simulink model "ACFTsim"  (R2024b)
settings: Solver=ode1  StartTime=0.0  StopTime=inf  FixedStep=0.01  RelTol=1e-3
model workspace (MAT data in the model file):
  op_trim1 = opcond.OperatingReport
  op_trim1.Outputs_(1) = opcond.OutputReport
  op_trim1.Outputs_(1).yspec_ = 0
  op_trim1.Outputs_(1).Block_ = 'ACFT/Mach'
  op_trim1.Outputs_(1).PortWidth_ = 1
  op_trim1.Outputs_(1).PortNumber_ = NaN
  op_trim1.Outputs_(1).y_ = 0.293890617808
  op_trim1.Outputs_(1).Known_ = 0
  op_trim1.Outputs_(1).Min_ = -Inf
  op_trim1.Outputs_(1).Max_ = Inf
  op_trim1.Outputs_(2) = opcond.OutputReport
  op_trim1.Outputs_(2).yspec_ = 0
  op_trim1.Outputs_(2).Block_ = 'ACFT/Beta_deg'
  op_trim1.Outputs_(2).PortWidth_ = 1
  op_trim1.Outputs_(2).PortNumber_ = NaN
  op_trim1.Outputs_(2).Known_ = 1
  op_trim1.Outputs_(2).Min_ = -Inf
  op_trim1.Outputs_(2).Max_ = Inf
  op_trim1.Outputs_(3) = opcond.OutputReport
  op_trim1.Outputs_(3).yspec_ = 0
  op_trim1.Outputs_(3).Block_ = 'ACFT/Alpha_deg'
  op_trim1.Outputs_(3).PortWidth_ = 1
  op_trim1.Outputs_(3).PortNumber_ = NaN
  op_trim1.Outputs_(3).Known_ = 0
  op_trim1.Outputs_(3).Min_ = -Inf
  op_trim1.Outputs_(3).Max_ = Inf
  op_trim1.Outputs_(4) = opcond.OutputReport
  op_trim1.Outputs_(4).yspec_ = 200
  op_trim1.Outputs_(4).Block_ = 'ACFT/Cas_kt'
  op_trim1.Outputs_(4).PortWidth_ = 1
  op_trim1.Outputs_(4).PortNumber_ = NaN
  op_trim1.Outputs_(4).y_ = 194.38408042
  op_trim1.Outputs_(4).Known_ = 1
  op_trim1.Outputs_(4).Min_ = -Inf
  op_trim1.Outputs_(4).Max_ = Inf
  op_trim1.Outputs_(5) = opcond.OutputReport
  op_trim1.Outputs_(5).yspec_ = 0
  op_trim1.Outputs_(5).Block_ = 'ACFT/u_mps'
  op_trim1.Outputs_(5).PortWidth_ = 1
  op_trim1.Outputs_(5).PortNumber_ = NaN
  op_trim1.Outputs_(5).y_ = 100
  op_trim1.Outputs_(5).Known_ = 0
  op_trim1.Outputs_(5).Min_ = -Inf
  op_trim1.Outputs_(5).Max_ = Inf
  op_trim1.Outputs_(6) = opcond.OutputReport
  op_trim1.Outputs_(6).yspec_ = 0
  op_trim1.Outputs_(6).Block_ = 'ACFT/v_mps'
  op_trim1.Outputs_(6).PortWidth_ = 1
  op_trim1.Outputs_(6).PortNumber_ = NaN
  op_trim1.Outputs_(6).Known_ = 0
  op_trim1.Outputs_(6).Min_ = -Inf
  op_trim1.Outputs_(6).Max_ = Inf
  op_trim1.Outputs_(7) = opcond.OutputReport
  op_trim1.Outputs_(7).yspec_ = 0
  op_trim1.Outputs_(7).Block_ = 'ACFT/w_mps'
  op_trim1.Outputs_(7).PortWidth_ = 1
  op_trim1.Outputs_(7).PortNumber_ = NaN
  op_trim1.Outputs_(7).Known_ = 0
  op_trim1.Outputs_(7).Min_ = -Inf
  op_trim1.Outputs_(7).Max_ = Inf
  op_trim1.Outputs_(8) = opcond.OutputReport
  op_trim1.Outputs_(8).yspec_ = 0
  op_trim1.Outputs_(8).Block_ = 'ACFT/phi_deg'
  op_trim1.Outputs_(8).PortWidth_ = 1
  op_trim1.Outputs_(8).PortNumber_ = NaN
  op_trim1.Outputs_(8).Known_ = 0
  op_trim1.Outputs_(8).Min_ = -Inf
  op_trim1.Outputs_(8).Max_ = Inf
  op_trim1.Outputs_(9) = opcond.OutputReport
  op_trim1.Outputs_(9).yspec_ = 0
  op_trim1.Outputs_(9).Block_ = 'ACFT/theta_deg'
  op_trim1.Outputs_(9).PortWidth_ = 1
  op_trim1.Outputs_(9).PortNumber_ = NaN
  op_trim1.Outputs_(9).Known_ = 0
  op_trim1.Outputs_(9).Min_ = -Inf
  op_trim1.Outputs_(9).Max_ = Inf
  op_trim1.Outputs_(10) = opcond.OutputReport
  op_trim1.Outputs_(10).yspec_ = 0
  op_trim1.Outputs_(10).Block_ = 'ACFT/psi_deg'
  op_trim1.Outputs_(10).PortWidth_ = 1
  op_trim1.Outputs_(10).PortNumber_ = NaN
  op_trim1.Outputs_(10).Known_ = 0
  op_trim1.Outputs_(10).Min_ = -Inf
  op_trim1.Outputs_(10).Max_ = Inf
  op_trim1.Outputs_(11) = opcond.OutputReport
  op_trim1.Outputs_(11).yspec_ = 0
  op_trim1.Outputs_(11).Block_ = 'ACFT/p_radps'
  op_trim1.Outputs_(11).PortWidth_ = 1
  op_trim1.Outputs_(11).PortNumber_ = NaN
  op_trim1.Outputs_(11).Known_ = 0
  op_trim1.Outputs_(11).Min_ = -Inf
  op_trim1.Outputs_(11).Max_ = Inf
  op_trim1.Outputs_(12) = opcond.OutputReport
  op_trim1.Outputs_(12).yspec_ = 0
  op_trim1.Outputs_(12).Block_ = 'ACFT/q_radps'
  op_trim1.Outputs_(12).PortWidth_ = 1
  op_trim1.Outputs_(12).PortNumber_ = NaN
  op_trim1.Outputs_(12).Known_ = 0
  op_trim1.Outputs_(12).Min_ = -Inf
  op_trim1.Outputs_(12).Max_ = Inf
  op_trim1.Outputs_(13) = opcond.OutputReport
  op_trim1.Outputs_(13).yspec_ = 0
  op_trim1.Outputs_(13).Block_ = 'ACFT/r_radps'
  op_trim1.Outputs_(13).PortWidth_ = 1
  op_trim1.Outputs_(13).PortNumber_ = NaN
  op_trim1.Outputs_(13).Known_ = 0
  op_trim1.Outputs_(13).Min_ = -Inf
  op_trim1.Outputs_(13).Max_ = Inf
  op_trim1.Outputs_(14) = opcond.OutputReport
  op_trim1.Outputs_(14).yspec_ = 0
  op_trim1.Outputs_(14).Block_ = 'ACFT/x_m'
  op_trim1.Outputs_(14).PortWidth_ = 1
  op_trim1.Outputs_(14).PortNumber_ = NaN
  op_trim1.Outputs_(14).Known_ = 0
  op_trim1.Outputs_(14).Min_ = -Inf
  op_trim1.Outputs_(14).Max_ = Inf
  op_trim1.Outputs_(15) = opcond.OutputReport
  op_trim1.Outputs_(15).yspec_ = 0
  op_trim1.Outputs_(15).Block_ = 'ACFT/y_m'
  op_trim1.Outputs_(15).PortWidth_ = 1
  op_trim1.Outputs_(15).PortNumber_ = NaN
  op_trim1.Outputs_(15).Known_ = 0
  op_trim1.Outputs_(15).Min_ = -Inf
  op_trim1.Outputs_(15).Max_ = Inf
  op_trim1.Outputs_(16) = opcond.OutputReport
  op_trim1.Outputs_(16).yspec_ = 25000
  op_trim1.Outputs_(16).Block_ = 'ACFT/PressAlt_ft'
  op_trim1.Outputs_(16).PortWidth_ = 1
  op_trim1.Outputs_(16).PortNumber_ = NaN
  op_trim1.Outputs_(16).y_ = 0
  op_trim1.Outputs_(16).Known_ = 1
  op_trim1.Outputs_(16).Min_ = -Inf
  op_trim1.Outputs_(16).Max_ = Inf
  op_trim1.Outputs_(17) = opcond.OutputReport
  op_trim1.Outputs_(17).yspec_ = 0
  op_trim1.Outputs_(17).Block_ = 'ACFT/Gspeed_kt'
  op_trim1.Outputs_(17).PortWidth_ = 1
  op_trim1.Outputs_(17).PortNumber_ = NaN
  op_trim1.Outputs_(17).y_ = 194.384450923
  op_trim1.Outputs_(17).Known_ = 0
  op_trim1.Outputs_(17).Min_ = -Inf
  op_trim1.Outputs_(17).Max_ = Inf
  op_trim1.Outputs_(18) = opcond.OutputReport
  op_trim1.Outputs_(18).yspec_ = 0
  op_trim1.Outputs_(18).Block_ = 'ACFT/Track_deg'
  op_trim1.Outputs_(18).PortWidth_ = 1
  op_trim1.Outputs_(18).PortNumber_ = NaN
  op_trim1.Outputs_(18).Known_ = 0
  op_trim1.Outputs_(18).Min_ = -Inf
  op_trim1.Outputs_(18).Max_ = Inf
  op_trim1.Outputs_(19) = opcond.OutputReport
  op_trim1.Outputs_(19).yspec_ = 0
  op_trim1.Outputs_(19).Block_ = 'ACFT/Gamma_deg'
  op_trim1.Outputs_(19).PortWidth_ = 1
  op_trim1.Outputs_(19).PortNumber_ = NaN
  op_trim1.Outputs_(19).y_ = 0
  op_trim1.Outputs_(19).Known_ = 1
  op_trim1.Outputs_(19).Min_ = -Inf
  op_trim1.Outputs_(19).Max_ = Inf
  op_trim1.Outputs_(20) = opcond.OutputReport
  op_trim1.Outputs_(20).yspec_ = 0
  op_trim1.Outputs_(20).Block_ = 'ACFT/nx'
  op_trim1.Outputs_(20).PortWidth_ = 1
  op_trim1.Outputs_(20).PortNumber_ = NaN
  op_trim1.Outputs_(20).y_ = -0.0431036960178
  op_trim1.Outputs_(20).Known_ = 0
  op_trim1.Outputs_(20).Min_ = -Inf
  op_trim1.Outputs_(20).Max_ = Inf
  op_trim1.Outputs_(21) = opcond.OutputReport
  op_trim1.Outputs_(21).yspec_ = 0
  op_trim1.Outputs_(21).Block_ = 'ACFT/ny'
  op_trim1.Outputs_(21).PortWidth_ = 1
  op_trim1.Outputs_(21).PortNumber_ = NaN
  op_trim1.Outputs_(21).Known_ = 0
  op_trim1.Outputs_(21).Min_ = -Inf
  op_trim1.Outputs_(21).Max_ = Inf
  op_trim1.Outputs_(22) = opcond.OutputReport
  op_trim1.Outputs_(22).yspec_ = 0
  op_trim1.Outputs_(22).Block_ = 'ACFT/nz'
  op_trim1.Outputs_(22).PortWidth_ = 1
  op_trim1.Outputs_(22).PortNumber_ = NaN
  op_trim1.Outputs_(22).y_ = 0.0431036960178
  op_trim1.Outputs_(22).Known_ = 0
  op_trim1.Outputs_(22).Min_ = -Inf
  op_trim1.Outputs_(22).Max_ = Inf
  op_trim1.Outputs_(23) = opcond.OutputReport
  op_trim1.Outputs_(23).yspec_ = 0
  op_trim1.Outputs_(23).Block_ = 'ACFT/Thrust_N'
  op_trim1.Outputs_(23).PortWidth_ = 1
  op_trim1.Outputs_(23).PortNumber_ = NaN
  op_trim1.Outputs_(23).Known_ = 0
  op_trim1.Outputs_(23).Min_ = -Inf
  op_trim1.Outputs_(23).Max_ = Inf
  op_trim1.Outputs_(24) = opcond.OutputReport
  op_trim1.Outputs_(24).yspec_ = 0
  op_trim1.Outputs_(24).Block_ = 'ACFT/Alpha_radps'
  op_trim1.Outputs_(24).PortWidth_ = 1
  op_trim1.Outputs_(24).PortNumber_ = NaN
  op_trim1.Outputs_(24).Known_ = 0
  op_trim1.Outputs_(24).Min_ = -Inf
  op_trim1.Outputs_(24).Max_ = Inf
  op_trim1.Outputs_(25) = opcond.OutputReport
  op_trim1.Outputs_(25).yspec_ = 0
  op_trim1.Outputs_(25).Block_ = 'ACFT/Tas_kt'
  op_trim1.Outputs_(25).PortWidth_ = 1
  op_trim1.Outputs_(25).PortNumber_ = NaN
  op_trim1.Outputs_(25).y_ = 194.384450923
  op_trim1.Outputs_(25).Known_ = 0
  op_trim1.Outputs_(25).Min_ = -Inf
  op_trim1.Outputs_(25).Max_ = Inf
  op_trim1.TerminationString_ = 'Could not find a solution that satisfies all constraints.  Relax the constraints to find a feasible solution.'
  op_trim1.OptimizationOutput_.iterations = 1
  op_trim1.OptimizationOutput_.funcCount = 16
  op_trim1.OptimizationOutput_.lssteplength = 1
  op_trim1.OptimizationOutput_.stepsize = 0
  op_trim1.OptimizationOutput_.algorithm = 'active-set'
  op_trim1.OptimizationOutput_.firstorderopt = []
  op_trim1.OptimizationOutput_.constrviolation = 25000
  op_trim1.OptimizationOutput_.message = 'Converged to an infeasible point.
    | 
    | fmincon stopped because the size of the current search direction is less than
    | twice the value of the step size tolerance but constraints are not 
    | satisfied to within the value of the constraint tolerance.
    | 
    | <stopping criteria details>
    | 
    | Optimization stopped because the norm of the current search direction , 0.000000e+00,
    | is less than 2*options.StepTolerance = 1.000000e-06, but the maximum constraint
    | violation, 2.500000e+04, exceeds options.ConstraintTolerance = 1.000000e-06.'
  op_trim1.OptimizationOutput_.bestfeasible = []
  op_trim1.OptimizationOutput_.progress = {'<font face="monospaced"; size=3><BR>', 'Optimizing to solve for all desired dx/dt=0, x(k+1)-x(k)=0, and y=ydes.<BR>', ' <BR>', '(Maximum Error)  Block<BR>', ' ---------------------------------------------------------<BR>', '(2.50000e+04) ACFT/PressAlt_ft<BR>', '(2.50000e+04) ACFT/PressAlt_ft<BR>', ' <BR>', 'Could not find a solution that satisfies all constraints.  Relax the constraints to find a feasible solution.<BR>'}
  op_trim1.Model_ = 'ACFT'
  op_trim1.States_(1) = opcond.StateReport
  op_trim1.States_(1).Nx_ = 1
  op_trim1.States_(1).Block_ = 'ACFT/EquationsMotions/BodyRates/p_radps'
  op_trim1.States_(1).SteadyState_ = 1
  op_trim1.States_(1).dxMin_ = -Inf
  op_trim1.States_(1).dxMax_ = Inf
  op_trim1.States_(1).Known_ = 0
  op_trim1.States_(1).Min_ = -Inf
  op_trim1.States_(1).Max_ = Inf
  op_trim1.States_(2) = opcond.StateReport
  op_trim1.States_(2).dx_ = 0.0213648728432
  op_trim1.States_(2).Nx_ = 1
  op_trim1.States_(2).Block_ = 'ACFT/EquationsMotions/BodyRates/q_radps'
  op_trim1.States_(2).SteadyState_ = 1
  op_trim1.States_(2).dxMin_ = -Inf
  op_trim1.States_(2).dxMax_ = Inf
  op_trim1.States_(2).Known_ = 0
  op_trim1.States_(2).Min_ = -Inf
  op_trim1.States_(2).Max_ = Inf
  op_trim1.States_(3) = opcond.StateReport
  op_trim1.States_(3).Nx_ = 1
  op_trim1.States_(3).Block_ = 'ACFT/EquationsMotions/BodyRates/r_radps'
  op_trim1.States_(3).SteadyState_ = 1
  op_trim1.States_(3).dxMin_ = -Inf
  op_trim1.States_(3).dxMax_ = Inf
  op_trim1.States_(3).Known_ = 0
  op_trim1.States_(3).Min_ = -Inf
  op_trim1.States_(3).Max_ = Inf
  op_trim1.States_(4) = opcond.StateReport
  op_trim1.States_(4).dx_ = -0.422702860553
  op_trim1.States_(4).Nx_ = 1
  op_trim1.States_(4).Block_ = 'ACFT/EquationsMotions/BodyVelocities/u_mps'
  op_trim1.States_(4).x_ = 100
  op_trim1.States_(4).SteadyState_ = 1
  op_trim1.States_(4).dxMin_ = -Inf
  op_trim1.States_(4).dxMax_ = Inf
  op_trim1.States_(4).Known_ = 1
  op_trim1.States_(4).Min_ = -Inf
  op_trim1.States_(4).Max_ = Inf
  op_trim1.States_(5) = opcond.StateReport
  op_trim1.States_(5).Nx_ = 1
  op_trim1.States_(5).Block_ = 'ACFT/EquationsMotions/BodyVelocities/v_mps'
  op_trim1.States_(5).SteadyState_ = 1
  op_trim1.States_(5).dxMin_ = -Inf
  op_trim1.States_(5).dxMax_ = Inf
  op_trim1.States_(5).Known_ = 0
  op_trim1.States_(5).Min_ = -Inf
  op_trim1.States_(5).Max_ = Inf
  op_trim1.States_(6) = opcond.StateReport
  op_trim1.States_(6).dx_ = 9.38394713945
  op_trim1.States_(6).Nx_ = 1
  op_trim1.States_(6).Block_ = 'ACFT/EquationsMotions/BodyVelocities/w_mps'
  op_trim1.States_(6).SteadyState_ = 1
  op_trim1.States_(6).dxMin_ = -Inf
  op_trim1.States_(6).dxMax_ = Inf
  op_trim1.States_(6).Known_ = 0
  op_trim1.States_(6).Min_ = -Inf
  op_trim1.States_(6).Max_ = Inf
  op_trim1.States_(7) = opcond.StateReport
  op_trim1.States_(7).dx_ = 100
  op_trim1.States_(7).Nx_ = 1
  op_trim1.States_(7).Block_ = 'ACFT/EquationsMotions/InertialData/XI_m'
  op_trim1.States_(7).SteadyState_ = 0
  op_trim1.States_(7).dxMin_ = -Inf
  op_trim1.States_(7).dxMax_ = Inf
  op_trim1.States_(7).Known_ = 0
  op_trim1.States_(7).Min_ = -Inf
  op_trim1.States_(7).Max_ = Inf
  op_trim1.States_(8) = opcond.StateReport
  op_trim1.States_(8).Nx_ = 1
  op_trim1.States_(8).Block_ = 'ACFT/EquationsMotions/InertialData/YI_m'
  op_trim1.States_(8).SteadyState_ = 0
  op_trim1.States_(8).dxMin_ = -Inf
  op_trim1.States_(8).dxMax_ = Inf
  op_trim1.States_(8).Known_ = 0
  op_trim1.States_(8).Min_ = -Inf
  op_trim1.States_(8).Max_ = Inf
  op_trim1.States_(9) = opcond.StateReport
  op_trim1.States_(9).Nx_ = 1
  op_trim1.States_(9).Block_ = 'ACFT/EquationsMotions/InertialData/ZI_m'
  op_trim1.States_(9).SteadyState_ = 0
  op_trim1.States_(9).dxMin_ = -Inf
  op_trim1.States_(9).dxMax_ = Inf
  op_trim1.States_(9).Known_ = 0
  op_trim1.States_(9).Min_ = -Inf
  op_trim1.States_(9).Max_ = Inf
  op_trim1.States_(10) = opcond.StateReport
  op_trim1.States_(10).Nx_ = 1
  op_trim1.States_(10).Block_ = 'ACFT/EquationsMotions/LBE_EulerAngles_rad/PHI_rad'
  op_trim1.States_(10).SteadyState_ = 1
  op_trim1.States_(10).dxMin_ = -Inf
  op_trim1.States_(10).dxMax_ = Inf
  op_trim1.States_(10).Known_ = 0
  op_trim1.States_(10).Min_ = -Inf
  op_trim1.States_(10).Max_ = Inf
  op_trim1.States_(11) = opcond.StateReport
  op_trim1.States_(11).Nx_ = 1
  op_trim1.States_(11).Block_ = 'ACFT/EquationsMotions/LBE_EulerAngles_rad/PSI_rad'
  op_trim1.States_(11).SteadyState_ = 1
  op_trim1.States_(11).dxMin_ = -Inf
  op_trim1.States_(11).dxMax_ = Inf
  op_trim1.States_(11).Known_ = 0
  op_trim1.States_(11).Min_ = -Inf
  op_trim1.States_(11).Max_ = Inf
  op_trim1.States_(12) = opcond.StateReport
  op_trim1.States_(12).Nx_ = 1
  op_trim1.States_(12).Block_ = 'ACFT/EquationsMotions/LBE_EulerAngles_rad/THETA_rad'
  op_trim1.States_(12).SteadyState_ = 1
  op_trim1.States_(12).dxMin_ = -Inf
  op_trim1.States_(12).dxMax_ = Inf
  op_trim1.States_(12).Known_ = 0
  op_trim1.States_(12).Min_ = -Inf
  op_trim1.States_(12).Max_ = Inf
  op_trim1.Inputs_(1) = opcond.InputReport
  op_trim1.Inputs_(1).Block_ = 'ACFT/Mass_kg'
  op_trim1.Inputs_(1).PortWidth_ = 1
  op_trim1.Inputs_(1).PortDimensions_ = [1 1]
  op_trim1.Inputs_(1).u_ = 15000
  op_trim1.Inputs_(1).Known_ = 1
  op_trim1.Inputs_(1).Min_ = -Inf
  op_trim1.Inputs_(1).Max_ = Inf
  op_trim1.Inputs_(2) = opcond.InputReport
  op_trim1.Inputs_(2).Block_ = 'ACFT/Elevator_deg'
  op_trim1.Inputs_(2).PortWidth_ = 1
  op_trim1.Inputs_(2).PortDimensions_ = [1 1]
  op_trim1.Inputs_(2).Known_ = 0
  op_trim1.Inputs_(2).Min_ = -30
  op_trim1.Inputs_(2).Max_ = 30
  op_trim1.Inputs_(3) = opcond.InputReport
  op_trim1.Inputs_(3).Block_ = 'ACFT/CG_mac'
  op_trim1.Inputs_(3).PortWidth_ = 1
  op_trim1.Inputs_(3).PortDimensions_ = [1 1]
  op_trim1.Inputs_(3).u_ = 0.4
  op_trim1.Inputs_(3).Known_ = 1
  op_trim1.Inputs_(3).Min_ = -Inf
  op_trim1.Inputs_(3).Max_ = Inf
  op_trim1.Inputs_(4) = opcond.InputReport
  op_trim1.Inputs_(4).Block_ = 'ACFT/Throttle_deg'
  op_trim1.Inputs_(4).PortWidth_ = 1
  op_trim1.Inputs_(4).PortDimensions_ = [1 1]
  op_trim1.Inputs_(4).Known_ = 0
  op_trim1.Inputs_(4).Min_ = 0
  op_trim1.Inputs_(4).Max_ = 1
  op_trim1.Inputs_(5) = opcond.InputReport
  op_trim1.Inputs_(5).Block_ = 'ACFT/Rudder_deg'
  op_trim1.Inputs_(5).PortWidth_ = 1
  op_trim1.Inputs_(5).PortDimensions_ = [1 1]
  op_trim1.Inputs_(5).Known_ = 0
  op_trim1.Inputs_(5).Min_ = -30
  op_trim1.Inputs_(5).Max_ = 30
  op_trim1.Inputs_(6) = opcond.InputReport
  op_trim1.Inputs_(6).Block_ = 'ACFT/Wind_x'
  op_trim1.Inputs_(6).PortWidth_ = 1
  op_trim1.Inputs_(6).PortDimensions_ = [1 1]
  op_trim1.Inputs_(6).Known_ = 1
  op_trim1.Inputs_(6).Min_ = -Inf
  op_trim1.Inputs_(6).Max_ = Inf
  op_trim1.Inputs_(7) = opcond.InputReport
  op_trim1.Inputs_(7).Block_ = 'ACFT/Wind_z'
  op_trim1.Inputs_(7).PortWidth_ = 1
  op_trim1.Inputs_(7).PortDimensions_ = [1 1]
  op_trim1.Inputs_(7).Known_ = 1
  op_trim1.Inputs_(7).Min_ = -Inf
  op_trim1.Inputs_(7).Max_ = Inf
  op_trim1.Inputs_(8) = opcond.InputReport
  op_trim1.Inputs_(8).Block_ = 'ACFT/Wind_y'
  op_trim1.Inputs_(8).PortWidth_ = 1
  op_trim1.Inputs_(8).PortDimensions_ = [1 1]
  op_trim1.Inputs_(8).Known_ = 1
  op_trim1.Inputs_(8).Min_ = -Inf
  op_trim1.Inputs_(8).Max_ = Inf
  op_trim1.Inputs_(9) = opcond.InputReport
  op_trim1.Inputs_(9).Block_ = 'ACFT/Aileron_deg'
  op_trim1.Inputs_(9).PortWidth_ = 1
  op_trim1.Inputs_(9).PortDimensions_ = [1 1]
  op_trim1.Inputs_(9).Known_ = 0
  op_trim1.Inputs_(9).Min_ = -40
  op_trim1.Inputs_(9).Max_ = 40
  op_trim4 : opcond.OperatingReport (value not decoded)
  u_mps = 0
values from neighbouring files (symbols this model uses):
  alfa_deg = -1.8    [initACFT_high.m]    (also in init_Cessna.m = 1)
  b = params.b    [Aerodynamics_Coefficient.m]    (also in AeroforcesandMoments.m; ConversionStab2Aero.m = dynP_Pa*CnB; initACFT_high.m = 21; initACFT_low.m = 21)
  c = params.c    [Aerodynamics_Coefficient.m]    (also in AeroforcesandMoments.m; ConversionStab2Aero.m = dynP_Pa*CmB; initACFT_high.m = 2.5; initACFT_low.m = 2.5)
  CD0 = params.CD0    [Aerodynamics_Coefficient.m]    (also in initACFT_high.m = 0.0281; initACFT_low.m = 0.023; init_Cessna.m = 0.027)
  CD_alpha = params.CD_alpha    [Aerodynamics_Coefficient.m]    (also in initACFT_high.m = 0.5157; initACFT_low.m = 0.1318; init_Cessna.m = 0.26)
  CD_elev = params.CD_elev    [Aerodynamics_Coefficient.m]    (also in initACFT_high.m = 0.0178; initACFT_low.m = 0.0178; init_Cessna.m = 0)
  CL0 = params.CL0    [Aerodynamics_Coefficient.m]    (also in initACFT_high.m = 0.209; initACFT_low.m = 0.19; init_Cessna.m = 0.307)
  Cl_ail = -0.0453    [initACFT_high.m]    (also in initACFT_low.m = -0.0516; init_Cessna.m = -0.229)
  CL_alpha = params.CL_alpha    [Aerodynamics_Coefficient.m]    (also in initACFT_high.m = 8.7491; initACFT_low.m = 6.1879; init_Cessna.m = 4.41)
  CL_AlphaDot = params.CL_AlphaDot    [Aerodynamics_Coefficient.m]    (also in initACFT_high.m = 1.27; initACFT_low.m = 1.93; init_Cessna.m = 0)
  Cl_beta = -0.1352    [initACFT_high.m]    (also in initACFT_low.m; init_Cessna.m = -0.0923)
  CL_elev = params.CL_elev    [Aerodynamics_Coefficient.m]    (also in initACFT_high.m = 0.538; initACFT_low.m = 0.4727; init_Cessna.m = 0.43)
  Cl_p = -0.45    [initACFT_high.m]    (also in initACFT_low.m; init_Cessna.m = -0.484)
  CL_q = params.CL_q    [Aerodynamics_Coefficient.m]    (also in initACFT_high.m = 4.14; initACFT_low.m = 4.66; init_Cessna.m = 3.9)
  Cl_r = 0.100    (= 0.1)    [initACFT_high.m]    (also in initACFT_low.m; init_Cessna.m = 0.0798)
  Cl_rud = 0.0333    [initACFT_high.m]    (also in initACFT_low.m = 0.0289; init_Cessna.m = 0.0147)
  Cm0 = params.Cm0    [Aerodynamics_Coefficient.m]    (also in initACFT_high.m = 0; initACFT_low.m = 0.0133; init_Cessna.m = 0.04)
  Cm_alpha = params.Cm_alpha    [Aerodynamics_Coefficient.m]    (also in initACFT_high.m = -2.4351; initACFT_low.m = -2.0168; init_Cessna.m = -0.613)
  Cm_AlphaDot = params.Cm_AlphaDot    [Aerodynamics_Coefficient.m]    (also in initACFT_high.m = -4.53; initACFT_low.m = -6.76; init_Cessna.m = -7.27)
  Cm_elev = params.Cm_elev    [Aerodynamics_Coefficient.m]    (also in initACFT_high.m = -1.9079; initACFT_low.m = -1.6788; init_Cessna.m = -1.122)
  Cm_q = params.Cm_q    [Aerodynamics_Coefficient.m]    (also in initACFT_high.m = -37.6; initACFT_low.m = -36.3; init_Cessna.m = -12.4)
  Cn_ail = -8.5944e-04    (= -0.00085944)    [initACFT_high.m]    (also in initACFT_low.m = -0.00063025; init_Cessna.m = -0.0216)
  Cn_beta = 0.1478    [initACFT_high.m]    (also in initACFT_low.m = 0.1209; init_Cessna.m = 0.0587)
  Cn_p = -0.114    [initACFT_high.m]    (also in initACFT_low.m; init_Cessna.m = -0.0278)
  Cn_r = -0.15    [initACFT_high.m]    (also in initACFT_low.m = -0.3; init_Cessna.m = -0.0937)
  Cn_rud = -0.1100    (= -0.11)    [initACFT_high.m]    (also in initACFT_low.m = -0.102; init_Cessna.m = -0.0645)
  CY_ail = 0    [initACFT_high.m]    (also in initACFT_low.m; init_Cessna.m)
  CY_beta = params.CY_beta    [Aerodynamics_Coefficient.m]    (also in initACFT_high.m = -1.2777; initACFT_low.m = -1.1803; init_Cessna.m = -0.404)
  CY_p = params.CY_p    [Aerodynamics_Coefficient.m]    (also in initACFT_high.m = 0.3; initACFT_low.m = 0.3; init_Cessna.m = -0.075)
  CY_r = params.CY_r    [Aerodynamics_Coefficient.m]    (also in initACFT_high.m = 0.91; initACFT_low.m = 0.91; init_Cessna.m = 0.214)
  CY_rud = params.CY_rud    [Aerodynamics_Coefficient.m]    (also in initACFT_high.m = 0.4343; initACFT_low.m = 0.4016; init_Cessna.m = 0.187)
  g = params.g_mps    [IsaAtmo.m]    (also in extForces.AndMoments.m = params.g; initACFT_high.m = 9.80665; init_Cessna.m = 9.80665)
  Inertia = [Ixx 0 -Ixz; 0 Iyy 0; -Ixz 0 Izz]    [initACFT_high.m]    (also in initACFT_low.m; init_Cessna.m)
  nrho = 0.75    [initACFT_high.m]    (also in initACFT_low.m; init_Cessna.m)
  nv = params.nv    [Propulsion.m]    (also in initACFT_high.m = 0; initACFT_low.m = 0; init_Cessna.m = -1)
  rho_reference_kgpm3 = 1.225    [initACFT_high.m]    (also in init_Cessna.m)
  S = 45    [initACFT_high.m]    (also in initACFT_low.m; init_Cessna.m = 16.2)
  Tmax = params.Tmax    [Propulsion.m]    (also in initACFT_high.m = 68000; initACFT_low.m = 68000; init_Cessna.m = 2070)
  Trimming = 0    [Sim_trim_input.m]    (also in init_Cessna.m)
  V_reference_mps = params.V    [Propulsion.m]    (also in initACFT_high.m = 200; init_Cessna.m = 51.4)
  xf_m = params.xf_m    [Propulsion.m]    (also in initACFT_high.m = -3.8; initACFT_low.m = -3.8; init_Cessna.m = 1)
  y_cg = 0    [initACFT_high.m]    (also in initACFT_low.m; init_Cessna.m)
  z_cg = -0.4    [initACFT_high.m]    (also in initACFT_low.m; init_Cessna.m = 0.2)
  zf_m = params.zf_m    [Propulsion.m]    (also in initACFT_high.m = -0.6; initACFT_low.m = -0.6; init_Cessna.m = 0)
undefined symbols (not defined in the file or in its folder): Earth, Receive, Send, WGS84
libraries: aerolibfltsims x2, vrlib x1, aerolibtransform2 x1
settings Model: PacingRate=0.110000  LastModifiedBy=jogos
settings DataIOCC: ExternalInput=getinputstruct(op_trim4)  InitialState=getstatestruct(op_trim4)

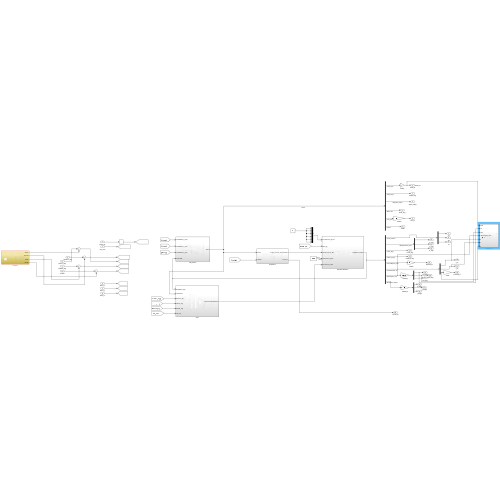
[thumbnail: Simulink's stored preview of the top-level diagram]
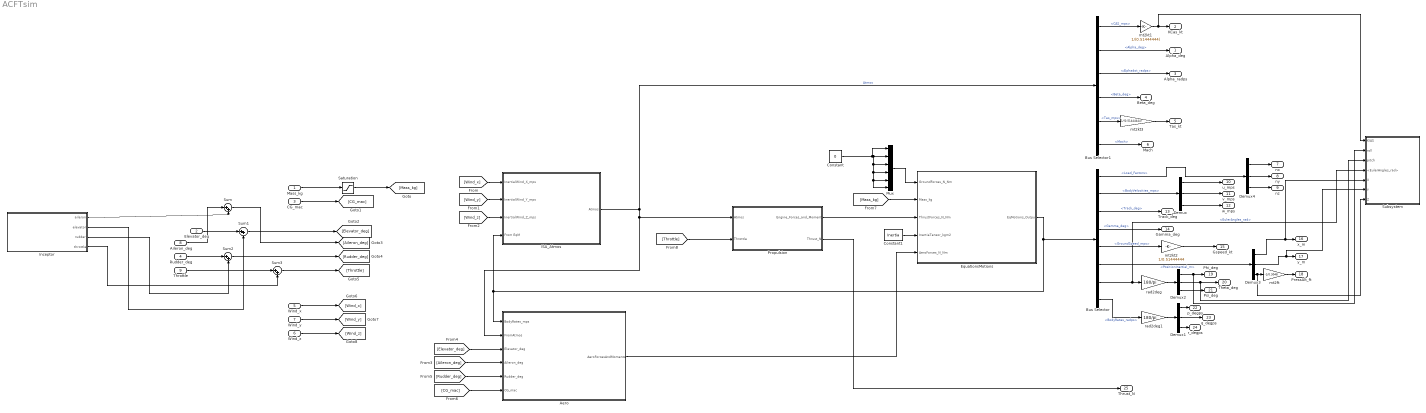
== system ACFTsim ==
  Mass_kg : Inport
  Elevator_deg : Inport  Port=2
  CG_mac : Inport  Port=3
  Rudder_deg : Inport  Port=4
  Wind_x : Inport  Port=5
  Wind_z : Inport  Port=6
  Wind_y : Inport  Port=7
  Aileron_deg : Inport  Port=8
  Throttle : Inport  Port=9
  Aero : Subsystem
  Bus Selector : BusSelector  OutputSignals=Load_Factors,BodyVelocities_mps,Track_deg,Gamma_deg,GroundSpeed_mps,PositionInertial_m,EulerAngles_rad,BodyRates_radps
  Bus Selector1 : BusSelector  OutputSignals=CAS_mps,Alpha_deg,Alphadot_radps,Beta_deg,Tas_mps,Mach
  Constant : Constant  Value=0
  Constant1 : Constant  Value=Inertia
  Demux{,1..4} (5 alike) : Demux  Outputs=3
  EquationsMotions : Subsystem
  ISA_Atmos : Subsystem
  Inceptor : Subsystem
  Mux : Mux  Inputs=6
  Propulsion : Subsystem
  Saturation : Saturate  UpperLimit=inf  LowerLimit=0.1
  Subsystem : Subsystem
  Sum{,1..3} (4 alike) : Sum  Inputs=|++
  mt2ft : Gain  Gain=-1/0.3048
  mt2kt1 : Gain  Gain=1/(0.51444444)
  mt2kt2 : Gain  Gain=1/0.51444444
  mt2kt3 : Gain  Gain=1/(0.51444444)
  rad2deg : Gain  Gain=180/pi
  rad2deg1 : Gain  Gain=180/pi
  Alpha_deg : Outport
  KCas_kt : Outport  Port=2  SignalName=KCas_kt
  Alpha_radps : Outport  Port=3
  Beta_deg : Outport  Port=4
  Tas_kt : Outport  Port=5
  Mach : Outport  Port=6
  nx : Outport  Port=7
  ny : Outport  Port=8
  nz : Outport  Port=9
  u_mps : Outport  Port=10
  v_mps : Outport  Port=11
  w_mps : Outport  Port=12
  Track_deg : Outport  Port=13
  Gamma_deg : Outport  Port=14
  Gspeed_kt : Outport  Port=15
  x_m : Outport  Port=16
  y_m : Outport  Port=17
  PressAlt_ft : Outport  Port=18
  Phi_deg : Outport  Port=19
  Theta_deg : Outport  Port=20
  Psi_deg : Outport  Port=21
  p_degps : Outport  Port=22
  q_degps : Outport  Port=23
  r_degps : Outport  Port=24
  Thrust_N : Outport  Port=25
  wires:
  EquationsMotions/1(EqMotions_Output) -> Aero/1(BodyRates_mps), ISA_Atmos/4(From EqM), Bus Selector/1
  ISA_Atmos/1(Atmos) -> Aero/2(FromAtmos), Propulsion/1(Atmos), Bus Selector1/1  "Atmos"
  Aero/1(AeroForcesAndMoments) -> EquationsMotions/5(AeroForces_N_Nm)
  Constant/1 -> Mux/1, Mux/6, Mux/5, Mux/4, Mux/3, Mux/2
  Mux/1 -> EquationsMotions/1(GroundForces_N_Nm)
  Constant1/1 -> EquationsMotions/4(InertiaTensor_kgm2)
  CG_mac/1 -> [CG_mac]
  Wind_x/1 -> [Wind_x]
  Wind_y/1 -> [Wind_y]
  Wind_z/1 -> [Wind_z]
  Mass_kg/1 -> Saturation/1
  [Wind_x] -> ISA_Atmos/1(InertialWind_X_mps)
  [Wind_y] -> ISA_Atmos/2(InertialWind_Y_mps)
  [Wind_z] -> ISA_Atmos/3(InertialWind_Z_mps)
  [Aileron_deg] -> Aero/4(Aileron_deg)
  [Elevator_deg] -> Aero/3(Elevator_deg)
  [Rudder_deg] -> Aero/5(Rudder_deg)
  [CG_mac] -> Aero/6(CG_mac)
  [Mass_kg] -> EquationsMotions/2(Mass_kg)
  Bus Selector1/1 -> mt2kt1/1  "<CAS_mps>"
  Bus Selector1/3 -> Alpha_radps/1  "<Alphadot_radps>"
  Bus Selector1/2 -> Alpha_deg/1  "<Alpha_deg>"
  Bus Selector1/4 -> Beta_deg/1  "<Beta_deg>"
  Bus Selector1/5 -> mt2kt3/1  "<Tas_mps>"
  Bus Selector1/6 -> Mach/1  "<Mach>"
  mt2kt1/1 -> Subsystem/1(KIAS), KCas_kt/1
  Bus Selector/2 -> Demux/1  "<BodyVelocities_mps>"
  Bus Selector/3 -> Track_deg/1  "<Track_deg>"
  Bus Selector/4 -> Gamma_deg/1  "<Gamma_deg>"
  Bus Selector/6 -> Demux3/1  "<PositionInertial_m>"
  Bus Selector/7 -> Subsystem/4(<EulerAngles_rad>), rad2deg/1  "<EulerAngles_rad>"
  Bus Selector/8 -> rad2deg1/1  "<BodyRates_radps>"
  rad2deg/1 -> Demux2/1
  rad2deg1/1 -> Demux1/1
  Demux/1 -> u_mps/1
  Demux/3 -> w_mps/1
  Demux/2 -> v_mps/1
  Demux2/2 -> Subsystem/3(pitch), Theta_deg/1
  Demux2/1 -> Subsystem/2(roll), Phi_deg/1
  Demux2/3 -> Psi_deg/1
  Demux1/1 -> p_degps/1
  Demux1/3 -> r_degps/1
  Demux1/2 -> q_degps/1
  Demux3/2 -> Subsystem/6(Y), y_m/1
  Demux3/1 -> Subsystem/5(X), x_m/1
  Demux3/3 -> Subsystem/7(Z), mt2ft/1
  mt2ft/1 -> PressAlt_ft/1
  Bus Selector/5 -> mt2kt2/1  "<GroundSpeed_mps>"
  mt2kt2/1 -> Gspeed_kt/1
  Bus Selector/1 -> Demux4/1  "<Load_Factors>"
  Demux4/1 -> nx/1
  Demux4/3 -> nz/1
  Demux4/2 -> ny/1
  Saturation/1 -> [Mass_kg]
  mt2kt3/1 -> Tas_kt/1
  Propulsion/1(Engine_Forces_and_Moments) -> EquationsMotions/3(ThrustForces_N_Nm)
  Propulsion/2(Thrust_N) -> Thrust_N/1
  [Throttle] -> Propulsion/2(Throttle)
  Inceptor/3(rudder) -> Sum2/2
  Inceptor/4(throttle) -> Sum3/2
  Inceptor/1(aileron) -> Sum/2
  Aileron_deg/1 -> Sum/1
  Sum/1 -> [Aileron_deg]
  Elevator_deg/1 -> Sum1/1
  Inceptor/2(elevator) -> Sum1/2
  Sum1/1 -> [Elevator_deg]
  Rudder_deg/1 -> Sum2/1
  Sum2/1 -> [Rudder_deg]
  Throttle/1 -> Sum3/1
  Sum3/1 -> [Throttle]

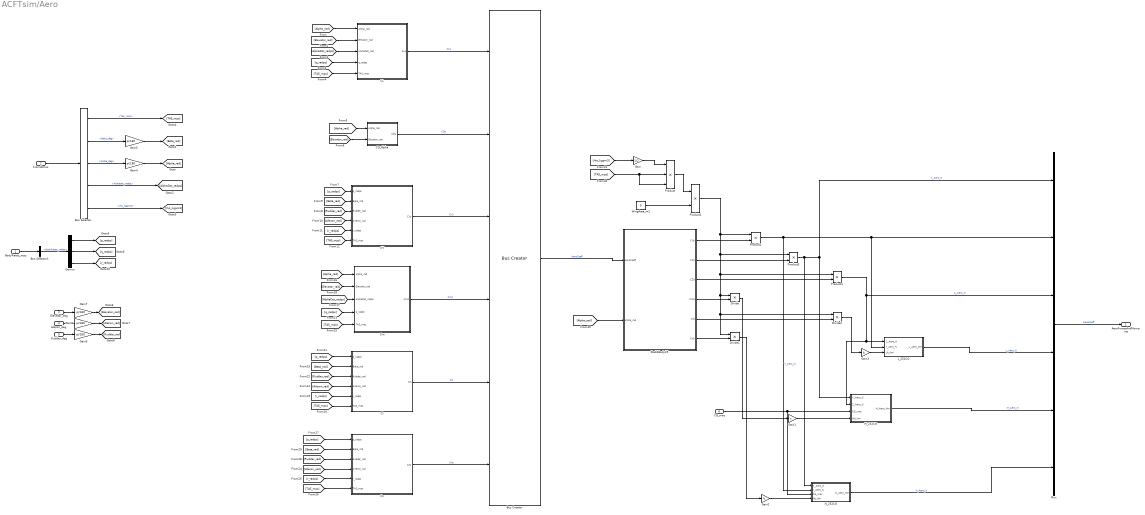
== system ACFTsim/Aero ==
  BodyRates_mps : Inport
  FromAtmos : Inport  Port=2
  Elevator_deg : Inport  Port=3
  Aileron_deg : Inport  Port=4
  Rudder_deg : Inport  Port=5
  CG_mac : Inport  Port=6
  Bus Creator : BusCreator  Inputs=6
  Bus Selector : BusSelector  OutputSignals=Tas_mps,Beta_deg,Alpha_deg,Alphadot_radps,rho_kgpm3
  Bus Selector1 : BusSelector  OutputSignals=BodyRates_radps
  CD_Alpha : Subsystem
  CI : Subsystem
  CL : Subsystem
  CY : Subsystem
  Cm : Subsystem
  Cn : Subsystem
  Demux : Demux  Outputs=3
  Divide : Product
  Divide1 : Product
  Divide2 : Product
  Gain : Gain  Gain=1/2
  Gain1 : Gain  Gain=c
  Gain2 : Gain  Gain=b
  Gain3 : Gain  Gain=b
  Gain{4..5,7..9} (5 alike) : Gain  Gain=pi/180
  L_252CG : Subsystem
  M_252CG : Subsystem
  Mux : Mux  Inputs=6
  N_252CG : Subsystem
  Product : Product  Inputs=3
  Product{1..4} (4 alike) : Product
  Stab2Body25 : Subsystem
  WingArea_m2 : Constant  Value=S
  AeroForcesAndMoments : Outport
  wires:
  [p_radps] -> Cn/1(p_radps)
  [r_radps] -> CI/5(r_radps)
  [rho_kgpm3] -> Gain/1
  Gain7/1 -> [Elevator_rad]
  CL/1(CLs) -> Bus Creator/1  "CLs"
  [TAS_mps] -> Cn/6(TAS_mps)
  [AlphaDot_radps] -> CL/3(AlphaDot_rad)
  N_252CG/1(N_Aero_Nm) -> Mux/6  "N_Aero_N"
  CI/1(CIs) -> Bus Creator/5  "CIs"
  M_252CG/1(M_Aero_Nm) -> Mux/5  "M_Aero_N"
  [p_radps] -> CY/1(p_radps)
  Stab2Body25/3(CZb) -> Product4/2
  [Alpha_rad] -> CL/1(Alpha_rad)
  [Aileron_rad] -> CI/4(Aileron_rad)
  Gain5/1 -> [Beta_rad]
  Cm/1(Cms) -> Bus Creator/4  "Cms"
  Gain2/1 -> N_252CG/4(Nb_Nm)
  [Beta_rad] -> CY/2(Beta_rad)
  Product2/1 -> N_252CG/2(Y_Aero_N), Mux/2, L_252CG/2(Y_Aero_N)  "Y_Aero_N"
  Elevator_deg/1 -> Gain7/1
  Gain/1 -> Product/1
  [Aileron_rad] -> Cn/4(Aileron_rad)
  CG_mac/1 -> N_252CG/3(CG_mac), M_252CG/3(CG_mac)
  [Rudder_rad] -> Cn/3(Rudder_rad)
  Demux/2 -> [q_radps]
  CD_Alpha/1(CDs) -> Bus Creator/2  "CDs"
  Demux/1 -> [p_radps]
  [TAS_mps] -> Cm/5(TAS_mps)
  [TAS_mps] -> Product/2, Product/3
  L_252CG/1(L_Aero_Nm) -> Mux/4  "L_Aero_N"
  Demux/3 -> [r_radps]
  CY/1(CYs) -> Bus Creator/3  "CYs"
  [AlphaDot_radps] -> Cm/3(AlphaDot_radps)
  [Rudder_rad] -> CI/3(Rudder_rad)
  [p_radps] -> CI/1(p_radps)
  [Rudder_rad] -> CY/3(Rudder_rad)
  Product1/1 -> Divide1/1, Divide2/1, Divide/1, Product4/1, Product3/1, Product2/1
  Gain1/1 -> M_252CG/4(Mb_Nm)
  Product4/1 -> L_252CG/1(Z_Aero_N), M_252CG/2(Z_Aero_N), Mux/3  "Z_Aero_N"
  [Elevator_rad] -> Cm/2(Elevator_rad)
  Gain9/1 -> [Rudder_rad]
  Aileron_deg/1 -> Gain8/1
  [Alpha_rad] -> Cm/1(Alpha_rad)
  Gain8/1 -> [Aileron_rad]
  [Beta_rad] -> Cn/2(Beta_rad)
  [Elevator_rad] -> CD_Alpha/2(Elevator_rad)
  Stab2Body25/1(CYb) -> Product2/2
  Rudder_deg/1 -> Gain9/1
  [Elevator_rad] -> CL/2(Elevator_rad)
  [Alpha_rad] -> Stab2Body25/2(Alpha_rad)
  Gain4/1 -> [Alpha_rad]
  Bus Creator/1 -> Stab2Body25/1(AeroCoeff)  "AeroCoeff"
  Stab2Body25/6(Cnb) -> Divide1/2
  Cn/1(Cns) -> Bus Creator/6  "Cns"
  WingArea_m2/1 -> Product1/2
  [Aileron_rad] -> CY/4(Aileron_rad)
  [TAS_mps] -> CL/5(TAS_mps)
  Product/1 -> Product1/1
  Stab2Body25/2(CXb) -> Product3/2
  [Alpha_rad] -> CD_Alpha/1(Alpha_rad)
  Product3/1 -> M_252CG/1(X_Aero_N), Mux/1, N_252CG/1(X_Aero_N)  "X_Aero_N"
  [Beta_rad] -> CI/2(Beta_rad)
  [TAS_mps] -> CI/6(TAS_mps)
  [r_radps] -> CY/5(r_radps)
  Mux/1 -> AeroForcesAndMoments/1  "AeroCoeff"
  Divide1/1 -> Gain2/1
  [q_radps] -> Cm/4(q_radps)
  [TAS_mps] -> CY/6(TAS_mps)
  Divide/1 -> Gain1/1
  [r_radps] -> Cn/5(r_radps)
  [q_radps] -> CL/4(q_radps)
  FromAtmos/1 -> Bus Selector/1
  Bus Selector/2 -> Gain5/1  "<Beta_deg>"
  Bus Selector/3 -> Gain4/1  "<Alpha_deg>"
  Bus Selector/4 -> [AlphaDot_radps]  "<Alphadot_radps>"
  Bus Selector/5 -> [rho_kgpm3]  "<rho_kgpm3>"
  Bus Selector/1 -> [TAS_mps]  "<Tas_mps>"
  BodyRates_mps/1 -> Bus Selector1/1
  Bus Selector1/1 -> Demux/1  "<BodyRates_radps>"
  Divide2/1 -> Gain3/1
  Gain3/1 -> L_252CG/3(Lb_Nm)
  Stab2Body25/5(Clb) -> Divide2/2
  Stab2Body25/4(Cmb) -> Divide/2

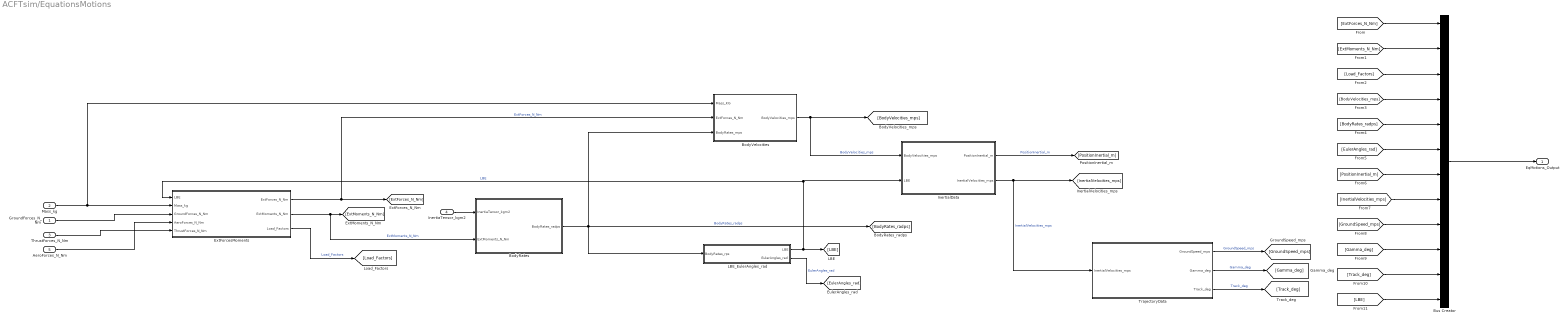
== system ACFTsim/EquationsMotions ==
  GroundForces_N_Nm : Inport
  Mass_kg : Inport  Port=2
  ThrustForces_N_Nm : Inport  Port=3
  InertiaTensor_kgm2 : Inport  Port=4
  AeroForces_N_Nm : Inport  Port=5
  BodyRates : Subsystem
  BodyVelocities : Subsystem
  Bus Creator : BusCreator  Inputs=12
  ExtForcesMoments : Subsystem
  InertialData : Subsystem
  LBE_EulerAngles_rad : Subsystem
  TrajectoryData : Subsystem
  EqMotions_Output : Outport
  wires:
  [Track_deg] -> Bus Creator/11
  [InertialVelocities_mps] -> Bus Creator/8
  [GroundSpeed_mps] -> Bus Creator/9
  [EulerAngles_rad] -> Bus Creator/6
  TrajectoryData/1(GroundSpeed_mps) -> [GroundSpeed_mps]  "GroundSpeed_mps"
  [Gamma_deg] -> Bus Creator/10
  TrajectoryData/2(Gamma_deg) -> [Gamma_deg]  "Gamma_deg"
  [ExtForces_N_Nm] -> Bus Creator/1
  TrajectoryData/3(Track_deg) -> [Track_deg]  "Track_deg"
  ExtForcesMoments/3(Load_Factors) -> [Load_Factors]  "Load_Factors"
  LBE_EulerAngles_rad/2(EulerAngles_rad) -> [EulerAngles_rad]  "EulerAngles_rad"
  InertialData/2(InertialVelocities_mps) -> TrajectoryData/1(InertialVelocities_mps), [InertialVelocities_mps]  "InertialVelocities_mps"
  [ExtMoments_N_Nm] -> Bus Creator/2
  BodyVelocities/1(BodyVelocities_mps) -> [BodyVelocities_mps], InertialData/1(BodyVelocities_mps)  "BodyVelocities_mps"
  ExtForcesMoments/2(ExtMoments_N_Nm) -> [ExtMoments_N_Nm], BodyRates/2(ExtMoments_N_Nm)  "ExtMoments_N_Nm"
  AeroForces_N_Nm/1 -> ExtForcesMoments/4(AeroForces_N_Nm)
  BodyRates/1(BodyRates_radps) -> LBE_EulerAngles_rad/1(BodyRates_rps), [BodyRates_radps], BodyVelocities/3(BodyRates_mps)  "BodyRates_radps"
  InertialData/1(PositionInertial_m) -> [PositionInertial_m]  "PositionInertial_m"
  Bus Creator/1 -> EqMotions_Output/1
  [BodyRates_radps] -> Bus Creator/5
  [PositionInertial_m] -> Bus Creator/7
  ThrustForces_N_Nm/1 -> ExtForcesMoments/5(ThrustForces_N_Nm)
  LBE_EulerAngles_rad/1(LBE) -> [LBE], InertialData/2(LBE), ExtForcesMoments/1(LBE)  "LBE"
  ExtForcesMoments/1(ExtForces_N_Nm) -> BodyVelocities/2(ExtForces_N_Nm), [ExtForces_N_Nm]  "ExtForces_N_Nm"
  [BodyVelocities_mps] -> Bus Creator/4
  InertiaTensor_kgm2/1 -> BodyRates/1(InertiaTensor_kgm2)
  GroundForces_N_Nm/1 -> ExtForcesMoments/3(GroundForces_N_Nm)
  Mass_kg/1 -> ExtForcesMoments/2(Mass_kg), BodyVelocities/1(Mass_KG)
  [Load_Factors] -> Bus Creator/3
  [LBE] -> Bus Creator/12

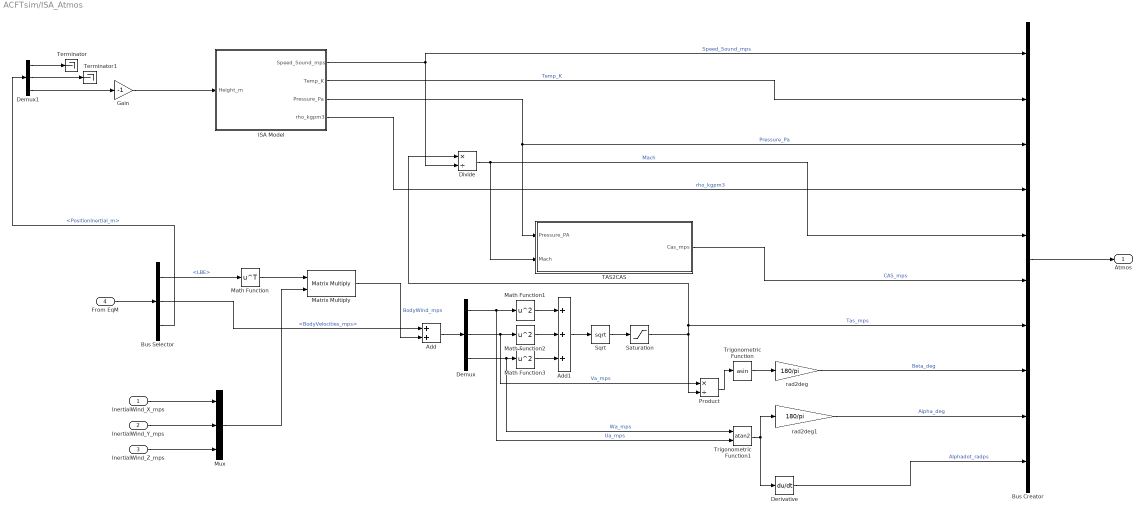
== system ACFTsim/ISA_Atmos ==
  InertialWind_X_mps : Inport
  InertialWind_Y_mps : Inport  Port=2
  InertialWind_Z_mps : Inport  Port=3
  From EqM : Inport  Port=4
  Add : Sum
  Add1 : Sum  Inputs=+++
  Bus Creator : BusCreator  Inputs=10
  Bus Selector : BusSelector  OutputSignals=LBE,BodyVelocities_mps,PositionInertial_m
  Demux : Demux  Outputs=3
  Demux1 : Demux  Outputs=3
  Derivative : Derivative
  Divide : Product  Inputs=*/
  Gain : Gain  Gain=-1
  ISA Model : Subsystem
  Math Function : Math  Operator=transpose
  Math Function1 : Math  Operator=square
  Math Function2 : Math  Operator=square
  Math Function3 : Math  Operator=square
  Matrix Multiply : Product  Multiplication=Matrix(*)
  Mux : Mux  Inputs=3
  Product : Product  Inputs=*/
  Saturation : Saturate  UpperLimit=inf  LowerLimit=0.1
  Sqrt : Sqrt
  TAS2CAS : Subsystem
  Terminator : Terminator
  Terminator1 : Terminator
  Trigonometric Function : Trigonometry  Operator=asin
  Trigonometric Function1 : Trigonometry  Operator=atan2
  rad2deg : Gain  Gain=180/pi
  rad2deg1 : Gain  Gain=180/pi
  Atmos : Outport
  wires:
  Matrix Multiply/1 -> Add/2  "BodyWind_mps"
  Add/1 -> Demux/1
  Add1/1 -> Sqrt/1
  Divide/1 -> TAS2CAS/2(Mach), Bus Creator/5  "Mach"
  rad2deg/1 -> Bus Creator/8  "Beta_deg"
  Demux/1 -> Trigonometric Function1/2, Math Function1/1  "Ua_mps"
  ISA Model/4(rho_kgpm3) -> Bus Creator/4  "rho_kgpm3"
  From EqM/1 -> Bus Selector/1
  TAS2CAS/1(Cas_mps) -> Bus Creator/6  "CAS_mps"
  Derivative/1 -> Bus Creator/10  "Alphadot_radps"
  Bus Creator/1 -> Atmos/1
  Mux/1 -> Matrix Multiply/2
  Math Function/1 -> Matrix Multiply/1
  Trigonometric Function1/1 -> rad2deg1/1, Derivative/1
  ISA Model/3(Pressure_Pa) -> Bus Creator/3, TAS2CAS/1(Pressure_PA)  "Pressure_Pa"
  Math Function3/1 -> Add1/3
  ISA Model/1(Speed_Sound_mps) -> Bus Creator/1, Divide/2  "Speed_Sound_mps"
  Sqrt/1 -> Saturation/1
  Math Function1/1 -> Add1/1
  ISA Model/2(Temp_K) -> Bus Creator/2  "Temp_K"
  Demux/3 -> Trigonometric Function1/1, Math Function3/1  "Wa_mps"
  Demux/2 -> Math Function2/1, Product/1  "Va_mps"
  Trigonometric Function/1 -> rad2deg/1
  InertialWind_X_mps/1 -> Mux/1
  Product/1 -> Trigonometric Function/1
  rad2deg1/1 -> Bus Creator/9  "Alpha_deg"
  Math Function2/1 -> Add1/2
  Bus Selector/1 -> Math Function/1  "<LBE>"
  Bus Selector/2 -> Add/1  "<BodyVelocities_mps>"
  Bus Selector/3 -> Demux1/1  "<PositionInertial_m>"
  Demux1/1 -> Terminator/1
  Demux1/2 -> Terminator1/1
  Demux1/3 -> Gain/1
  Gain/1 -> ISA Model/1(Height_m)
  Saturation/1 -> Divide/1, Bus Creator/7, Product/2  "Tas_mps"
  InertialWind_Y_mps/1 -> Mux/2
  InertialWind_Z_mps/1 -> Mux/3

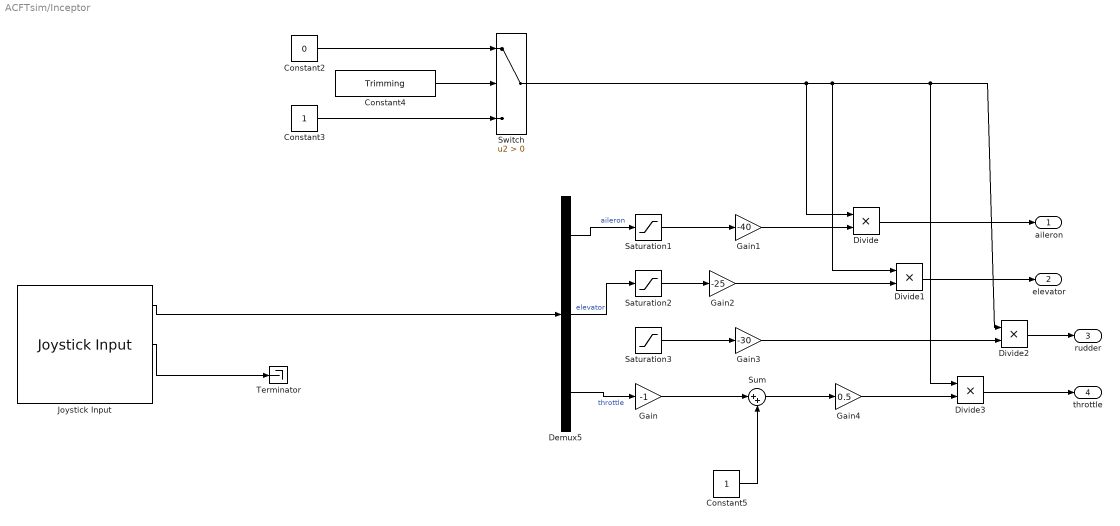
== system ACFTsim/Inceptor ==
  Constant2 : Constant  Value=0
  Constant3 : Constant
  Constant4 : Constant  Value=Trimming
  Constant5 : Constant
  Demux5 : Demux  Outputs=3
  Divide{,1..3} (4 alike) : Product  Inputs=**
  Gain : Gain  Gain=-1
  Gain1 : Gain  Gain=-40
  Gain2 : Gain  Gain=-25
  Gain3 : Gain  Gain=-30
  Gain4 : Gain  Gain=0.5
  Joystick Input : vrlib/Joystick Input  joyid=1  adjustports=on  forcefeed=off
  Saturation1 : Saturate  UpperLimit=inf  LowerLimit=0.1
  Saturation2 : Saturate  UpperLimit=inf  LowerLimit=0.1
  Saturation3 : Saturate  UpperLimit=inf  LowerLimit=0.1
  Sum : Sum  Inputs=|++
  Switch : Switch  Criteria=u2 > Threshold  SaturateOnIntegerOverflow=off  InputSameDT=off
  Terminator : Terminator
  aileron : Outport
  elevator : Outport  Port=2
  rudder : Outport  Port=3
  throttle : Outport  Port=4
  wires:
  Gain3/1 -> Divide2/2
  Demux5/1 -> Saturation1/1  "aileron"
  Constant2/1 -> Switch/1
  Sum/1 -> Gain4/1
  Switch/1 -> Divide/1, Divide3/1, Divide2/1, Divide1/1
  Divide3/1 -> throttle/1
  Gain2/1 -> Divide1/2
  Saturation1/1 -> Gain1/1
  Constant5/1 -> Sum/2
  Gain1/1 -> Divide/2
  Constant3/1 -> Switch/3
  Constant4/1 -> Switch/2
  Joystick Input/1 -> Demux5/1
  Saturation3/1 -> Gain3/1
  Demux5/2 -> Saturation2/1  "elevator"
  Joystick Input/2 -> Terminator/1
  Divide/1 -> aileron/1
  Saturation2/1 -> Gain2/1
  Gain/1 -> Sum/1
  Divide1/1 -> elevator/1
  Gain4/1 -> Divide3/2
  Divide2/1 -> rudder/1
  Demux5/3 -> Gain/1  "throttle"

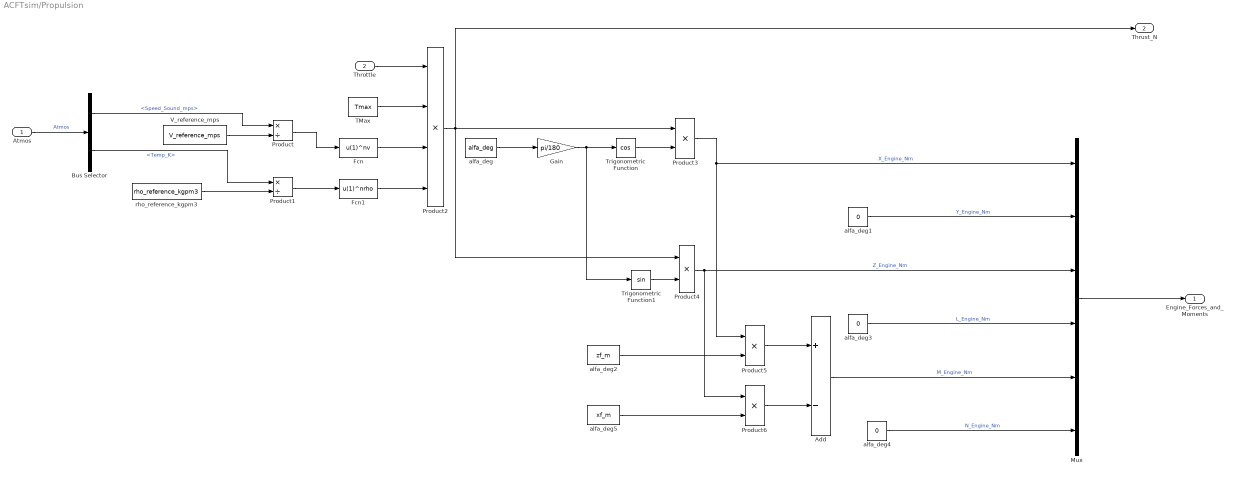
== system ACFTsim/Propulsion ==
  Atmos : Inport
  Throttle : Inport  Port=2
  Add : Sum  Inputs=+-
  Bus Selector : BusSelector  OutputSignals=Speed_Sound_mps,Temp_K
  Fcn : Fcn  Expr=u(1)^nv
  Fcn1 : Fcn  Expr=u(1)^nrho
  Gain : Gain  Gain=pi/180
  Mux : Mux  Inputs=6
  Product : Product  Inputs=*/
  Product1 : Product  Inputs=*/
  Product2 : Product  Inputs=****
  Product{3..6} (4 alike) : Product
  TMax : Constant  Value=Tmax
  Trigonometric Function : Trigonometry  Operator=cos
  Trigonometric Function1 : Trigonometry
  V_reference_mps : Constant  Value=V_reference_mps
  alfa_deg : Constant  Value=alfa_deg
  alfa_deg1 : Constant  Value=0
  alfa_deg2 : Constant  Value=zf_m
  alfa_deg3 : Constant  Value=0
  alfa_deg4 : Constant  Value=0
  alfa_deg5 : Constant  Value=xf_m
  rho_reference_kgpm3 : Constant  Value=rho_reference_kgpm3
  Engine_Forces_and_Moments : Outport
  Thrust_N : Outport  Port=2
  wires:
  alfa_deg/1 -> Gain/1
  alfa_deg1/1 -> Mux/2  "Y_Engine_Nm"
  Fcn/1 -> Product2/3
  Product3/1 -> Mux/1, Product5/1  "X_Engine_Nm"
  TMax/1 -> Product2/2
  alfa_deg3/1 -> Mux/4  "L_Engine_Nm"
  Trigonometric Function1/1 -> Product4/2
  Fcn1/1 -> Product2/4
  Add/1 -> Mux/5  "M_Engine_Nm"
  alfa_deg4/1 -> Mux/6  "N_Engine_Nm"
  Bus Selector/2 -> Product1/1  "<Temp_K>"
  Gain/1 -> Trigonometric Function/1, Trigonometric Function1/1
  Bus Selector/1 -> Product/1  "<Speed_Sound_mps>"
  Product1/1 -> Fcn1/1
  Atmos/1 -> Bus Selector/1  "Atmos"
  Product4/1 -> Mux/3, Product6/1  "Z_Engine_Nm"
  Product/1 -> Fcn/1
  Product2/1 -> Product3/1, Product4/1, Thrust_N/1
  rho_reference_kgpm3/1 -> Product1/2
  Product6/1 -> Add/2
  Product5/1 -> Add/1
  Mux/1 -> Engine_Forces_and_Moments/1
  V_reference_mps/1 -> Product/2
  alfa_deg2/1 -> Product5/2
  alfa_deg5/1 -> Product6/2
  Trigonometric Function/1 -> Product3/2
  Throttle/1 -> Product2/1

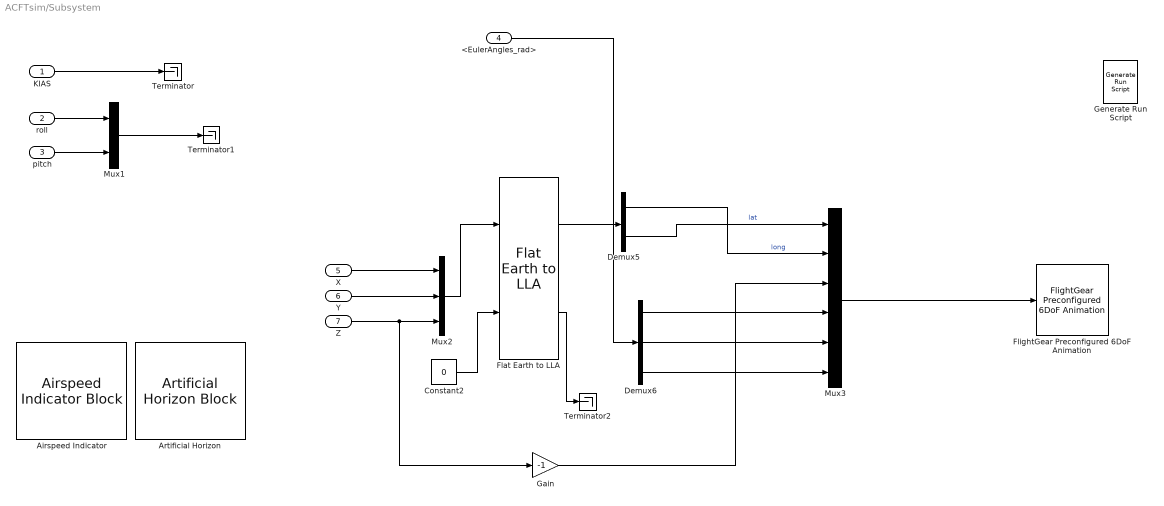
== system ACFTsim/Subsystem ==
  KIAS : Inport
  roll : Inport  Port=2
  pitch : Inport  Port=3
  <EulerAngles_rad> : Inport  Port=4
  X : Inport  Port=5
  Y : Inport  Port=6
  Z : Inport  Port=7
  Airspeed Indicator : AirspeedIndicatorBlock
  Artificial Horizon : ArtificialHorizonBlock
  Constant2 : Constant  Value=0
  Demux5 : Demux  Outputs=2
  Demux6 : Demux  Outputs=3
  Flat Earth to LLA : aerolibtransform2/Flat Earth to LLA  units=Metric (MKS)  ptype=Earth (WGS84)  F=1/298.257223563  R=6378137  refPosPort=off  LL0=[0 10]  psi=0
  FlightGear Preconfigured 6DoF Animation : aerolibfltsims/FlightGear Preconfigured 6DoF Animation  xFlightGearVersion=v2019.1  DestinationIpAddress=127.0.0.1  DestinationPort=5502  SampleTime=1/30  packetVersion=24
  Gain : Gain  Gain=-1
  Generate Run Script : aerolibfltsims/Generate Run Script  Architecture=Win64  dataFlow=Send-Receive  GeometryModelName=c172p  AirportId=KSFO  RunwayId=10L  InitialAltitude=7224  InitialHeading=113  OffsetDistance=4.72  OffsetAzimuth=0  InstallScenery=on  DisableShaders=off  OriginAddress=127.0.0.1  DestinationPort=5502  OriginPort=5505  LocalAddress=127.0.0.1  OutputFileName=runfg.bat  FlightGearBaseDirectory=C:\Program Files\FlightGear 2020.3
  Mux1 : Mux  Inputs=2
  Mux2 : Mux  Inputs=3
  Mux3 : Mux  Inputs=6
  Terminator : Terminator
  Terminator1 : Terminator
  Terminator2 : Terminator
  wires:
  <EulerAngles_rad>/1 -> Demux6/1
  Demux5/2 -> Mux3/1  "lat"
  Y/1 -> Mux2/2
  Mux1/1 -> Terminator1/1
  Demux6/2 -> Mux3/5
  Constant2/1 -> Flat Earth to LLA/2
  Demux6/1 -> Mux3/4
  pitch/1 -> Mux1/2
  X/1 -> Mux2/1
  Z/1 -> Gain/1, Mux2/3
  Flat Earth to LLA/1 -> Demux5/1
  Mux3/1 -> FlightGear Preconfigured 6DoF Animation/1
  roll/1 -> Mux1/1
  Gain/1 -> Mux3/3
  Demux5/1 -> Mux3/2  "long"
  KIAS/1 -> Terminator/1
  Demux6/3 -> Mux3/6
  Mux2/1 -> Flat Earth to LLA/1
  Flat Earth to LLA/2 -> Terminator2/1

== system ACFTsim/Aero/CD_Alpha ==
  Alpha_rad : Inport
  Elevator_rad : Inport  Port=2
  Abs : Abs  SaturateOnIntegerOverflow=off
  Abs1 : Abs  SaturateOnIntegerOverflow=off
  Add : Sum  Inputs=+++
  Constant : Constant  Value=CD0
  Gain : Gain  Gain=CD_alpha
  Gain1 : Gain  Gain=CD_elev
  CDs : Outport
  wires:
  Gain/1 -> Add/2
  Gain1/1 -> Add/3
  Elevator_rad/1 -> Abs1/1
  Add/1 -> CDs/1
  Abs/1 -> Gain/1
  Constant/1 -> Add/1
  Alpha_rad/1 -> Abs/1
  Abs1/1 -> Gain1/1

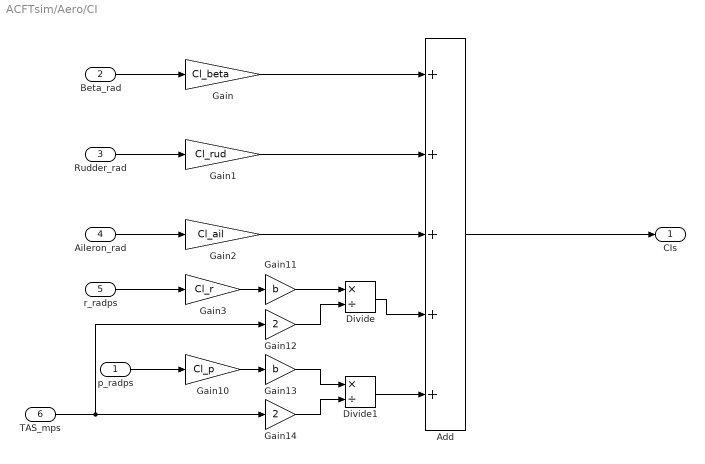
== system ACFTsim/Aero/CI ==
  p_radps : Inport
  Beta_rad : Inport  Port=2
  Rudder_rad : Inport  Port=3
  Aileron_rad : Inport  Port=4
  r_radps : Inport  Port=5
  TAS_mps : Inport  Port=6
  Add : Sum  Inputs=+++++
  Divide : Product  Inputs=*/
  Divide1 : Product  Inputs=*/
  Gain : Gain  Gain=Cl_beta
  Gain1 : Gain  Gain=Cl_rud
  Gain10 : Gain  Gain=Cl_p
  Gain11 : Gain  Gain=b
  Gain12 : Gain  Gain=2
  Gain13 : Gain  Gain=b
  Gain14 : Gain  Gain=2
  Gain2 : Gain  Gain=Cl_ail
  Gain3 : Gain  Gain=Cl_r
  CIs : Outport
  wires:
  Divide1/1 -> Add/5
  r_radps/1 -> Gain3/1
  Beta_rad/1 -> Gain/1
  Aileron_rad/1 -> Gain2/1
  Gain1/1 -> Add/2
  p_radps/1 -> Gain10/1
  Divide/1 -> Add/4
  Gain10/1 -> Gain13/1
  TAS_mps/1 -> Gain14/1, Gain12/1
  Gain14/1 -> Divide1/2
  Gain11/1 -> Divide/1
  Gain12/1 -> Divide/2
  Add/1 -> CIs/1
  Gain2/1 -> Add/3
  Rudder_rad/1 -> Gain1/1
  Gain3/1 -> Gain11/1
  Gain/1 -> Add/1
  Gain13/1 -> Divide1/1

== system ACFTsim/Aero/CL ==
  Alpha_rad : Inport
  Elevator_rad : Inport  Port=2
  AlphaDot_rad : Inport  Port=3
  q_radps : Inport  Port=4
  TAS_mps : Inport  Port=5
  Add : Sum  Inputs=+++++
  Constant : Constant  Value=CL0
  Divide : Product  Inputs=*/
  Divide1 : Product  Inputs=*/
  Gain : Gain  Gain=CL_alpha
  Gain1 : Gain  Gain=CL_elev
  Gain2 : Gain  Gain=CL_AlphaDot
  Gain3 : Gain  Gain=CL_q
  Gain4 : Gain  Gain=c
  Gain5 : Gain  Gain=2
  Gain6 : Gain  Gain=c
  Gain7 : Gain  Gain=2
  CLs : Outport
  wires:
  Gain7/1 -> Divide1/2
  Divide1/1 -> Add/4
  Gain6/1 -> Divide1/1
  Gain4/1 -> Divide/1
  Divide/1 -> Add/5
  Gain5/1 -> Divide/2
  TAS_mps/1 -> Gain5/1, Gain7/1
  Gain3/1 -> Gain4/1
  Add/1 -> CLs/1
  Gain2/1 -> Gain6/1
  Constant/1 -> Add/1
  Gain/1 -> Add/2
  Elevator_rad/1 -> Gain1/1
  Gain1/1 -> Add/3
  AlphaDot_rad/1 -> Gain2/1
  q_radps/1 -> Gain3/1
  Alpha_rad/1 -> Gain/1

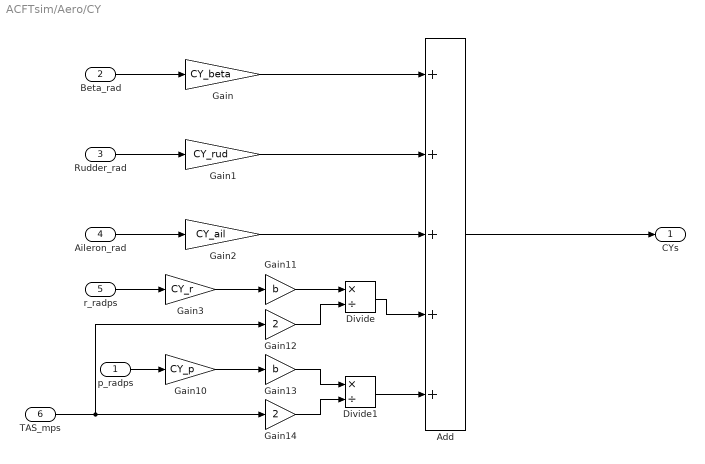
== system ACFTsim/Aero/CY ==
  p_radps : Inport
  Beta_rad : Inport  Port=2
  Rudder_rad : Inport  Port=3
  Aileron_rad : Inport  Port=4
  r_radps : Inport  Port=5
  TAS_mps : Inport  Port=6
  Add : Sum  Inputs=+++++
  Divide : Product  Inputs=*/
  Divide1 : Product  Inputs=*/
  Gain : Gain  Gain=CY_beta
  Gain1 : Gain  Gain=CY_rud
  Gain10 : Gain  Gain=CY_p
  Gain11 : Gain  Gain=b
  Gain12 : Gain  Gain=2
  Gain13 : Gain  Gain=b
  Gain14 : Gain  Gain=2
  Gain2 : Gain  Gain=CY_ail
  Gain3 : Gain  Gain=CY_r
  CYs : Outport
  wires:
  Divide1/1 -> Add/5
  r_radps/1 -> Gain3/1
  Beta_rad/1 -> Gain/1
  Aileron_rad/1 -> Gain2/1
  Gain1/1 -> Add/2
  p_radps/1 -> Gain10/1
  Divide/1 -> Add/4
  Gain10/1 -> Gain13/1
  TAS_mps/1 -> Gain14/1, Gain12/1
  Gain14/1 -> Divide1/2
  Gain11/1 -> Divide/1
  Gain12/1 -> Divide/2
  Add/1 -> CYs/1
  Gain2/1 -> Add/3
  Rudder_rad/1 -> Gain1/1
  Gain3/1 -> Gain11/1
  Gain/1 -> Add/1
  Gain13/1 -> Divide1/1

== system ACFTsim/Aero/Cm ==
  Alpha_rad : Inport
  Elevator_rad : Inport  Port=2
  AlphaDot_radps : Inport  Port=3
  q_radps : Inport  Port=4
  TAS_mps : Inport  Port=5
  Add : Sum  Inputs=+++++
  Constant : Constant  Value=Cm0
  Gain : Gain  Gain=Cm_alpha
  Gain1 : Gain  Gain=2
  Gain10 : Gain  Gain=Cm_AlphaDot
  Gain11 : Gain  Gain=c
  Gain12 : Gain  Gain=Cm_q
  Gain13 : Gain  Gain=2
  Gain2 : Gain  Gain=Cm_elev
  Gain3 : Gain  Gain=c
  Product : Product  Inputs=*/
  Product1 : Product  Inputs=*/
  Cms : Outport
  wires:
  Add/1 -> Cms/1
  Product/1 -> Add/4
  Gain/1 -> Add/2
  Gain11/1 -> Product1/1
  Gain10/1 -> Gain3/1
  q_radps/1 -> Gain12/1
  Gain12/1 -> Gain11/1
  Gain13/1 -> Product1/2
  Gain3/1 -> Product/1
  Product1/1 -> Add/5
  Alpha_rad/1 -> Gain/1
  Gain2/1 -> Add/3
  Gain1/1 -> Product/2
  TAS_mps/1 -> Gain13/1, Gain1/1
  Constant/1 -> Add/1
  Elevator_rad/1 -> Gain2/1
  AlphaDot_radps/1 -> Gain10/1

== system ACFTsim/Aero/Cn ==
  p_radps : Inport
  Beta_rad : Inport  Port=2
  Rudder_rad : Inport  Port=3
  Aileron_rad : Inport  Port=4
  r_radps : Inport  Port=5
  TAS_mps : Inport  Port=6
  Add : Sum  Inputs=+++++
  Divide : Product  Inputs=*/
  Divide1 : Product  Inputs=*/
  Gain : Gain  Gain=Cn_beta
  Gain1 : Gain  Gain=Cn_rud
  Gain10 : Gain  Gain=Cn_p
  Gain11 : Gain  Gain=b
  Gain12 : Gain  Gain=2
  Gain13 : Gain  Gain=b
  Gain14 : Gain  Gain=2
  Gain2 : Gain  Gain=Cn_ail
  Gain3 : Gain  Gain=Cn_r
  Cns : Outport
  wires:
  Divide1/1 -> Add/5
  r_radps/1 -> Gain3/1
  Beta_rad/1 -> Gain/1
  Aileron_rad/1 -> Gain2/1
  Gain1/1 -> Add/2
  p_radps/1 -> Gain10/1
  Divide/1 -> Add/4
  Gain10/1 -> Gain13/1
  TAS_mps/1 -> Gain14/1, Gain12/1
  Gain14/1 -> Divide1/2
  Gain11/1 -> Divide/1
  Gain12/1 -> Divide/2
  Add/1 -> Cns/1
  Gain2/1 -> Add/3
  Rudder_rad/1 -> Gain1/1
  Gain3/1 -> Gain11/1
  Gain/1 -> Add/1
  Gain13/1 -> Divide1/1

== system ACFTsim/Aero/L_252CG ==
  Z_Aero_N : Inport
  Y_Aero_N : Inport  Port=2
  Lb_Nm : Inport  Port=3
  Add : Sum  Inputs=--+
  Constant : Constant  Value=z_cg
  Product5 : Product
  Product6 : Product
  Y_cg_m : Constant  Value=y_cg
  L_Aero_Nm : Outport
  wires:
  Lb_Nm/1 -> Add/3
  Add/1 -> L_Aero_Nm/1  "L_Aero_Nm"
  Z_Aero_N/1 -> Product6/1
  Constant/1 -> Product5/2
  Y_Aero_N/1 -> Product5/1
  Y_cg_m/1 -> Product6/2
  Product5/1 -> Add/1
  Product6/1 -> Add/2

== system ACFTsim/Aero/M_252CG ==
  X_Aero_N : Inport
  Z_Aero_N : Inport  Port=2
  CG_mac : Inport  Port=3
  Mb_Nm : Inport  Port=4
  Add : Sum  Inputs=-++
  Fcn : Fcn  Expr=(u(1)-0.25)*c
  Product5 : Product
  Product6 : Product
  Z_cg_m : Constant  Value=z_cg
  M_Aero_Nm : Outport
  wires:
  Mb_Nm/1 -> Add/3
  Add/1 -> M_Aero_Nm/1  "M_Aero_Nm"
  X_Aero_N/1 -> Product6/1
  Fcn/1 -> Product5/2
  Z_Aero_N/1 -> Product5/1
  Z_cg_m/1 -> Product6/2
  Product5/1 -> Add/1
  CG_mac/1 -> Fcn/1
  Product6/1 -> Add/2

== system ACFTsim/Aero/N_252CG ==
  X_Aero_N : Inport
  Y_Aero_N : Inport  Port=2
  CG_mac : Inport  Port=3
  Nb_Nm : Inport  Port=4
  Add : Sum  Inputs=+++
  Fcn : Fcn  Expr=(u(1)-0.25)*c
  Product5 : Product
  Product6 : Product
  Y_cg_m : Constant  Value=y_cg
  N_Aero_Nm : Outport
  wires:
  Nb_Nm/1 -> Add/3
  Add/1 -> N_Aero_Nm/1  "N_Aero_Nm"
  X_Aero_N/1 -> Product6/1
  Fcn/1 -> Product5/2
  Y_Aero_N/1 -> Product5/1
  Y_cg_m/1 -> Product6/2
  Product5/1 -> Add/1
  CG_mac/1 -> Fcn/1
  Product6/1 -> Add/2

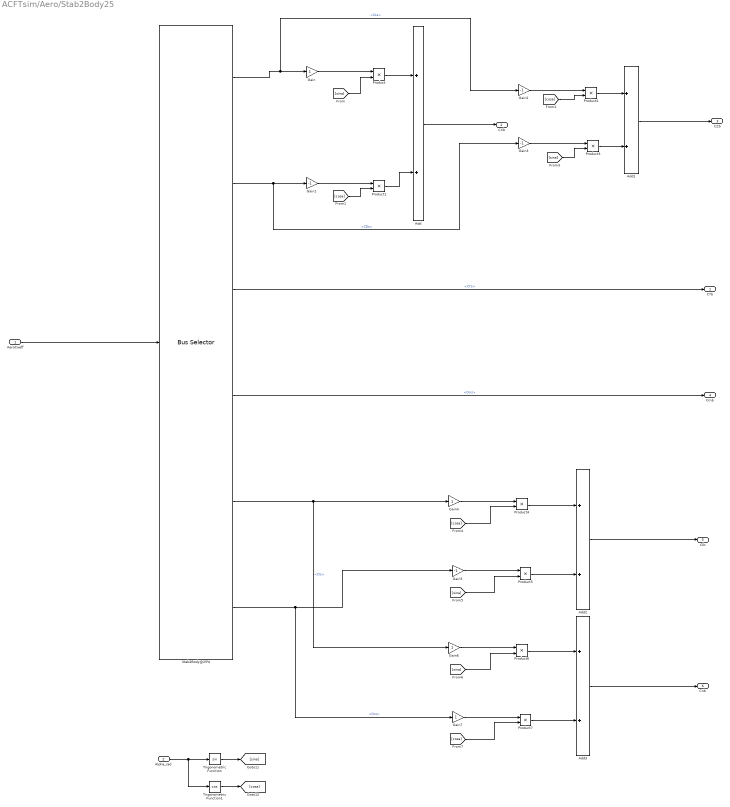
== system ACFTsim/Aero/Stab2Body25 ==
  AeroCoeff : Inport
  Alpha_rad : Inport  Port=2
  Add{,1..3} (4 alike) : Sum
  Gain{,4,6..7} (4 alike) : Gain
  Gain{1..3,5} (4 alike) : Gain  Gain=-1
  Product{,1..7} (8 alike) : Product
  Stab2Body@25% : BusSelector  OutputSignals=CLs,CDs,CYs,Cms,CIs,Cns
  Trigonometric Function : Trigonometry
  Trigonometric Function1 : Trigonometry  Operator=cos
  CYb : Outport
  CXb : Outport  Port=2
  CZb : Outport  Port=3
  Cmb : Outport  Port=4
  Clb : Outport  Port=5
  Cnb : Outport  Port=6
  wires:
  Stab2Body@25%/4 -> Cmb/1  "<Cms>"
  [sina] -> Product3/2
  Stab2Body@25%/2 -> Gain1/1, Gain3/1  "<CDs>"
  Gain2/1 -> Product2/1
  Product3/1 -> Add1/2
  Add1/1 -> CZb/1
  [cosa] -> Product2/2
  Gain3/1 -> Product3/1
  Product2/1 -> Add1/1
  Add/1 -> CXb/1
  [cosa] -> Product1/2
  [sina] -> Product/2
  Gain1/1 -> Product1/1
  Gain/1 -> Product/1
  Product1/1 -> Add/2
  Product/1 -> Add/1
  Alpha_rad/1 -> Trigonometric Function/1, Trigonometric Function1/1
  Trigonometric Function1/1 -> [cosa]
  Trigonometric Function/1 -> [sina]
  Stab2Body@25%/1 -> Gain/1, Gain2/1  "<CLs>"
  Stab2Body@25%/3 -> CYb/1  "<CYs>"
  AeroCoeff/1 -> Stab2Body@25%/1
  Gain4/1 -> Product4/1
  Product4/1 -> Add2/1
  Add2/1 -> Clb/1
  [cosa] -> Product4/2
  Gain5/1 -> Product5/1
  [sina] -> Product5/2
  Product5/1 -> Add2/2
  Stab2Body@25%/6 -> Gain7/1, Gain5/1  "<Cns>"
  [cosa] -> Product7/2
  Gain6/1 -> Product6/1
  [sina] -> Product6/2
  Product6/1 -> Add3/1
  Gain7/1 -> Product7/1
  Add3/1 -> Cnb/1
  Product7/1 -> Add3/2
  Stab2Body@25%/5 -> Gain6/1, Gain4/1  "<CIs>"

== system ACFTsim/EquationsMotions/BodyRates ==
  InertiaTensor_kgm2 : Inport
  ExtMoments_N_Nm : Inport  Port=2
  CrossProduct : Subsystem
  Demux : Demux  Outputs=3
  Mux : Mux  Inputs=3
  Product : Product  Multiplication=Matrix(*)
  Product1 : Product  Inputs=/*  Multiplication=Matrix(*)
  Sum : Sum  Inputs=-+
  p_radps : Integrator
  q_radps : Integrator
  r_radps : Integrator
  BodyRates_radps : Outport
  wires:
  Mux/1 -> CrossProduct/1(A), Product/2, BodyRates_radps/1  "BodyRates_radps"
  ExtMoments_N_Nm/1 -> Sum/2
  p_radps/1 -> Mux/1  "p_radps"
  CrossProduct/1(C) -> Sum/1
  InertiaTensor_kgm2/1 -> Product/1, Product1/1
  Product/1 -> CrossProduct/2(B)
  Sum/1 -> Product1/2
  Demux/1 -> p_radps/1
  q_radps/1 -> Mux/2  "q_radps"
  Demux/3 -> r_radps/1
  Demux/2 -> q_radps/1
  r_radps/1 -> Mux/3  "r_radps"
  Product1/1 -> Demux/1

== system ACFTsim/EquationsMotions/BodyVelocities ==
  Mass_KG : Inport
  ExtForces_N_Nm : Inport  Port=2
  BodyRates_mps : Inport  Port=3
  Add : Sum  Inputs=+-
  CrossProduct : Subsystem
  Demux : Demux  Outputs=3
  Mux : Mux  Inputs=3
  Product : Product  Inputs=*/
  u_mps : Integrator
  v_mps : Integrator
  w_mps : Integrator
  BodyVelocities_mps : Outport
  wires:
  BodyRates_mps/1 -> CrossProduct/1(A)
  v_mps/1 -> Mux/2
  Demux/2 -> v_mps/1
  u_mps/1 -> Mux/1
  Demux/3 -> w_mps/1
  Demux/1 -> u_mps/1
  Mux/1 -> BodyVelocities_mps/1, CrossProduct/2(B)  "BodyVelocities_mps"
  w_mps/1 -> Mux/3
  Product/1 -> Add/1
  Add/1 -> Demux/1  "BodyVelocitiesDot_mps"
  CrossProduct/1(C) -> Add/2
  ExtForces_N_Nm/1 -> Product/1
  Mass_KG/1 -> Product/2

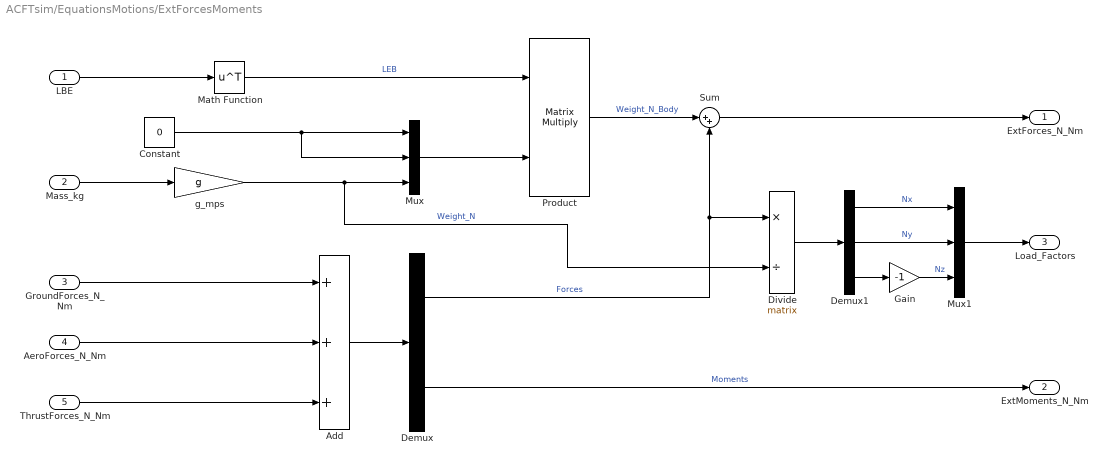
== system ACFTsim/EquationsMotions/ExtForcesMoments ==
  LBE : Inport
  Mass_kg : Inport  Port=2
  GroundForces_N_Nm : Inport  Port=3
  AeroForces_N_Nm : Inport  Port=4
  ThrustForces_N_Nm : Inport  Port=5
  Add : Sum  Inputs=+++
  Constant : Constant  Value=0
  Demux : Demux  Outputs=2
  Demux1 : Demux  Outputs=3
  Divide : Product  Inputs=*/  Multiplication=Matrix(*)
  Gain : Gain  Gain=-1
  Math Function : Math  Operator=transpose
  Mux : Mux  Inputs=3
  Mux1 : Mux  Inputs=3
  Product : Product  Multiplication=Matrix(*)
  Sum : Sum  Inputs=|++
  g_mps : Gain  Gain=g
  ExtForces_N_Nm : Outport
  ExtMoments_N_Nm : Outport  Port=2
  Load_Factors : Outport  Port=3
  wires:
  Demux1/2 -> Mux1/2  "Ny"
  Demux1/3 -> Gain/1
  AeroForces_N_Nm/1 -> Add/2
  g_mps/1 -> Divide/2, Mux/3  "Weight_N"
  Math Function/1 -> Product/1  "LEB"
  Mux/1 -> Product/2
  Gain/1 -> Mux1/3  "Nz"
  Mass_kg/1 -> g_mps/1
  ThrustForces_N_Nm/1 -> Add/3
  Sum/1 -> ExtForces_N_Nm/1
  LBE/1 -> Math Function/1
  Demux/1 -> Divide/1, Sum/2  "Forces"
  Constant/1 -> Mux/2, Mux/1
  Add/1 -> Demux/1
  Divide/1 -> Demux1/1
  GroundForces_N_Nm/1 -> Add/1
  Demux/2 -> ExtMoments_N_Nm/1  "Moments"
  Demux1/1 -> Mux1/1  "Nx"
  Mux1/1 -> Load_Factors/1
  Product/1 -> Sum/1  "Weight_N_Body"

== system ACFTsim/EquationsMotions/InertialData ==
  BodyVelocities_mps : Inport
  LBE : Inport  Port=2
  Demux : Demux  Outputs=3
  Matrix Multiply : Product  Multiplication=Matrix(*)
  Mux : Mux  Inputs=3
  XI_m : Integrator
  YI_m : Integrator
  ZI_m : Integrator
  PositionInertial_m : Outport
  InertialVelocities_mps : Outport  Port=2
  wires:
  Mux/1 -> PositionInertial_m/1  "PositionInertial_m"
  LBE/1 -> Matrix Multiply/1
  BodyVelocities_mps/1 -> Matrix Multiply/2
  Demux/2 -> YI_m/1
  YI_m/1 -> Mux/2
  ZI_m/1 -> Mux/3
  Matrix Multiply/1 -> Demux/1, InertialVelocities_mps/1  "InertialVelocities_mps"
  Demux/1 -> XI_m/1
  Demux/3 -> ZI_m/1
  XI_m/1 -> Mux/1

== system ACFTsim/EquationsMotions/LBE_EulerAngles_rad ==
  BodyRates_rps : Inport
  Demux : Demux  Outputs=3
  EulerRates_radps : Subsystem
  LBE_rotation : Subsystem
  Mux : Mux  Inputs=3
  PHI_rad : Integrator
  PSI_rad : Integrator
  THETA_rad : Integrator
  LBE : Outport
  EulerAngles_rad : Outport  Port=2
  wires:
  Mux/1 -> EulerAngles_rad/1, EulerRates_radps/2(EulerAngles_rad), LBE_rotation/1(EulerAngles_rad)  "EulerAngles_rad"
  EulerRates_radps/1(EulerRates_radps) -> Demux/1  "EulerRates_radps"
  BodyRates_rps/1 -> EulerRates_radps/1(BodyRates_rps)
  LBE_rotation/1(LBE) -> LBE/1
  Demux/3 -> PSI_rad/1
  Demux/1 -> PHI_rad/1
  THETA_rad/1 -> Mux/2
  PHI_rad/1 -> Mux/1
  PSI_rad/1 -> Mux/3
  Demux/2 -> THETA_rad/1

== system ACFTsim/EquationsMotions/TrajectoryData ==
  InertialVelocities_mps : Inport
  Add : Sum
  Demux : Demux  Outputs=3
  Gain : Gain  Gain=-1
  Gain1 : Gain  Gain=180/pi
  Gain2 : Gain  Gain=180/pi
  Math Function : Math  Operator=square
  Math Function1 : Math  Operator=square
  Sqrt : Sqrt
  Trigonometric Function : Trigonometry  Operator=atan2
  Trigonometric Function1 : Trigonometry  Operator=atan2
  GroundSpeed_mps : Outport
  Gamma_deg : Outport  Port=2
  Track_deg : Outport  Port=3
  wires:
  InertialVelocities_mps/1 -> Demux/1
  Trigonometric Function/1 -> Gain1/1
  Math Function1/1 -> Add/2
  Gain1/1 -> Gamma_deg/1
  Demux/2 -> Trigonometric Function1/1, Math Function1/1
  Demux/1 -> Trigonometric Function1/2, Math Function/1
  Gain2/1 -> Track_deg/1
  Gain/1 -> Trigonometric Function/1
  Math Function/1 -> Add/1
  Trigonometric Function1/1 -> Gain2/1
  Demux/3 -> Gain/1
  Sqrt/1 -> Trigonometric Function/2, GroundSpeed_mps/1
  Add/1 -> Sqrt/1

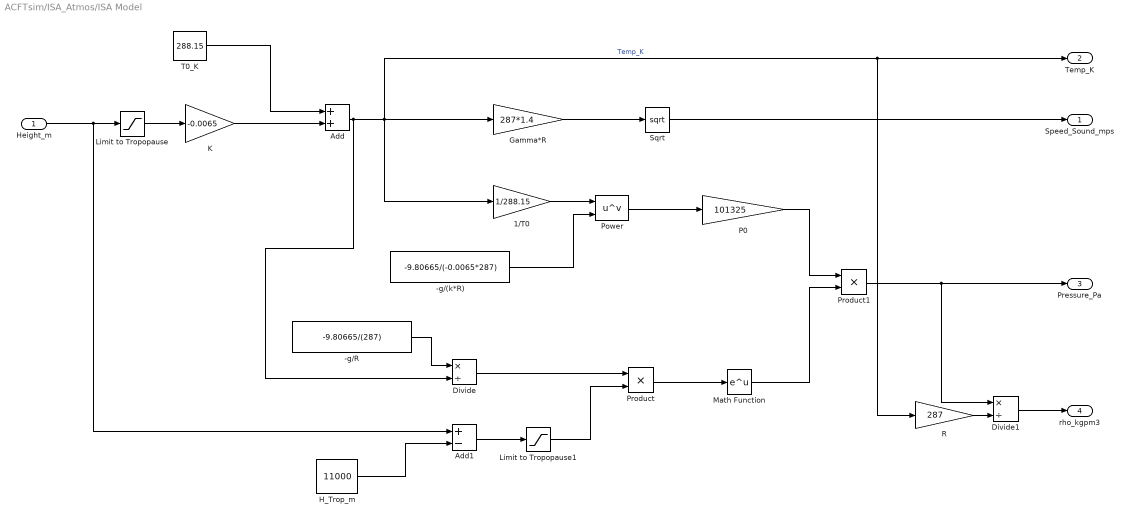
== system ACFTsim/ISA_Atmos/ISA Model ==
  Height_m : Inport
  -g/(k*R) : Constant  Value=-9.80665/(-0.0065*287)
  -g/R : Constant  Value=-9.80665/(287)
  1/T0 : Gain  Gain=1/288.15
  Add : Sum
  Add1 : Sum  Inputs=+-
  Divide : Product  Inputs=*/
  Divide1 : Product  Inputs=*/
  Gamma*R : Gain  Gain=287*1.4
  H_Trop_m : Constant  Value=11000
  K : Gain  Gain=-0.0065
  Limit to Tropopause : Saturate  UpperLimit=11000  LowerLimit=0
  Limit to Tropopause1 : Saturate  UpperLimit=inf  LowerLimit=0
  Math Function : Math
  P0 : Gain  Gain=101325
  Power : Math  Operator=pow  SignedPower=on
  Product : Product
  Product1 : Product
  R : Gain  Gain=287
  Sqrt : Sqrt
  T0_K : Constant  Value=288.15
  Speed_Sound_mps : Outport
  Temp_K : Outport  Port=2
  Pressure_Pa : Outport  Port=3
  rho_kgpm3 : Outport  Port=4
  wires:
  Product/1 -> Math Function/1
  Math Function/1 -> Product1/2
  Divide/1 -> Product/1
  P0/1 -> Product1/1
  K/1 -> Add/2
  Add/1 -> Divide/2, Gamma*R/1, 1/T0/1, Temp_K/1, R/1  "Temp_K"
  R/1 -> Divide1/2
  Divide1/1 -> rho_kgpm3/1
  Limit to Tropopause1/1 -> Product/2
  Product1/1 -> Divide1/1, Pressure_Pa/1
  Gamma*R/1 -> Sqrt/1
  H_Trop_m/1 -> Add1/2
  Add1/1 -> Limit to Tropopause1/1
  Sqrt/1 -> Speed_Sound_mps/1
  Height_m/1 -> Limit to Tropopause/1, Add1/1
  Power/1 -> P0/1
  -g/R/1 -> Divide/1
  Limit to Tropopause/1 -> K/1
  -g/(k*R)/1 -> Power/2
  1/T0/1 -> Power/1
  T0_K/1 -> Add/1

== system ACFTsim/ISA_Atmos/TAS2CAS ==
  Pressure_PA : Inport
  Mach : Inport  Port=2
  (Gamma-1)/2 : Gain  Gain=(1.4-1)/2
  (Gamma-1)/Gamma : Constant  Value=(1.4-1)/1.4
  2*(a0*a0)/(gamma-1) : Gain  Gain=(2*340.262^2)/(1.4-1)
  Add : Sum
  Add1 : Sum  Inputs=+-
  Add2 : Sum
  Add3 : Sum  Inputs=+-
  Constant : Constant
  Divide1 : Product  Inputs=*/
  Gamma/(Gamma-1) : Constant  Value=1.4/(1.4-1)
  Math Function : Math  Operator=square
  Math Function1 : Math  Operator=pow  SignedPower=on
  Math Function2 : Math  Operator=pow  SignedPower=on
  P0_Pa : Constant  Value=101325
  Product : Product
  Sqrt : Sqrt
  Cas_mps : Outport
  wires:
  2*(a0*a0)/(gamma-1)/1 -> Sqrt/1
  Mach/1 -> Math Function/1
  Product/1 -> Divide1/1
  Sqrt/1 -> Cas_mps/1
  Math Function1/1 -> Add1/1
  Add3/1 -> 2*(a0*a0)/(gamma-1)/1
  Math Function2/1 -> Add3/1
  (Gamma-1)/Gamma/1 -> Math Function2/2
  Divide1/1 -> Add2/1
  Constant/1 -> Add/2, Add3/2, Add2/2, Add1/2
  Add2/1 -> Math Function2/1
  P0_Pa/1 -> Divide1/2
  Gamma/(Gamma-1)/1 -> Math Function1/2
  Pressure_PA/1 -> Product/1
  Add/1 -> Math Function1/1
  Add1/1 -> Product/2
  (Gamma-1)/2/1 -> Add/1
  Math Function/1 -> (Gamma-1)/2/1

== system ACFTsim/EquationsMotions/BodyRates/CrossProduct ==
  A : Inport
  B : Inport  Port=2
  Add : Sum  Inputs=+-
  Demux : Demux  Outputs=3
  Demux1 : Demux  Outputs=3
  Mux : Mux  Inputs=3
  Mux1 : Mux  Inputs=3
  Product{,1..5} (6 alike) : Product
  C : Outport
  wires:
  Mux1/1 -> Add/2
  Add/1 -> C/1  "AxB"
  Product3/1 -> Mux1/1
  Product2/1 -> Mux/3
  Product1/1 -> Mux/2
  Mux/1 -> Add/1
  Product4/1 -> Mux1/2
  Product/1 -> Mux/1
  A/1 -> Demux/1
  B/1 -> Demux1/1
  Product5/1 -> Mux1/3
  Demux/2 -> Product5/1, Product/1
  Demux1/3 -> Product4/2, Product/2
  Demux/3 -> Product3/1, Product1/1
  Demux1/1 -> Product5/2, Product1/2
  Demux/1 -> Product4/1, Product2/1
  Demux1/2 -> Product3/2, Product2/2

== system ACFTsim/EquationsMotions/BodyVelocities/CrossProduct ==
  A : Inport
  B : Inport  Port=2
  Add : Sum  Inputs=+-
  Demux : Demux  Outputs=3
  Demux1 : Demux  Outputs=3
  Mux : Mux  Inputs=3
  Mux1 : Mux  Inputs=3
  Product{,1..5} (6 alike) : Product
  C : Outport
  wires:
  Mux1/1 -> Add/2
  Add/1 -> C/1  "AxB"
  Product3/1 -> Mux1/1
  Product2/1 -> Mux/3
  Product1/1 -> Mux/2
  Mux/1 -> Add/1
  Product4/1 -> Mux1/2
  Product/1 -> Mux/1
  A/1 -> Demux/1
  B/1 -> Demux1/1
  Product5/1 -> Mux1/3
  Demux/2 -> Product5/1, Product/1
  Demux1/3 -> Product4/2, Product/2
  Demux/3 -> Product3/1, Product1/1
  Demux1/1 -> Product5/2, Product1/2
  Demux/1 -> Product4/1, Product2/1
  Demux1/2 -> Product3/2, Product2/2

== system ACFTsim/EquationsMotions/LBE_EulerAngles_rad/EulerRates_radps ==
  BodyRates_rps : Inport
  EulerAngles_rad : Inport  Port=2
  Abs : Abs  SaturateOnIntegerOverflow=off
  Constant : Constant  Value=0.001
  Demux : Demux  Outputs=3
  Divide : Product  Inputs=**
  Mux : Mux  Inputs=3
  Mux1 : Mux  Inputs=3
  Mux2 : Mux  Inputs=3
  Relay : Relay  OnSwitchValue=0.001  OffSwitchValue=0  OnOutputValue=0  OffOutputValue=1
  Sign : Signum
  Switch : Switch  Criteria=u2 > Threshold  SaturateOnIntegerOverflow=off  InputSameDT=off
  Trigonometric Function : Trigonometry  Operator=sincos
  phidot_radps2 : Fcn  Expr=u(1)+u(2)*u(4)*(u(5)/u(8))+u(3)*u(7)*(u(5)/u(8))
  psidot_radps2 : Fcn  Expr=(u(2)*u(4)+u(3)*u(7))/u(8)
  thetadot_radps2 : Fcn  Expr=u(2)*u(7)-u(3)*u(4)
  EulerRates_radps : Outport
  wires:
  psidot_radps2/1 -> Mux1/3
  Abs/1 -> Relay/1
  Trigonometric Function/2 -> Demux/1
  Relay/1 -> Switch/2
  Mux2/1 -> Mux/3
  thetadot_radps2/1 -> Mux1/2
  Mux/1 -> psidot_radps2/1, thetadot_radps2/1, phidot_radps2/1
  phidot_radps2/1 -> Mux1/1
  Demux/2 -> Sign/1, Switch/3, Abs/1
  Switch/1 -> Mux2/2
  Sign/1 -> Divide/2
  Constant/1 -> Divide/1
  Mux1/1 -> EulerRates_radps/1
  EulerAngles_rad/1 -> Trigonometric Function/1
  Trigonometric Function/1 -> Mux/2
  Demux/1 -> Mux2/1
  BodyRates_rps/1 -> Mux/1
  Demux/3 -> Mux2/3
  Divide/1 -> Switch/1

== system ACFTsim/EquationsMotions/LBE_EulerAngles_rad/LBE_rotation ==
  EulerAngles_rad : Inport
  Fcn : Fcn  Expr=u(5)*u(6)
  Fcn1 : Fcn  Expr=u(1)*u(2)*u(6)-u(4)*u(3)
  Fcn2 : Fcn  Expr=u(6)*u(2)*u(4)+u(1)*u(3)
  Fcn3 : Fcn  Expr=u(5)*u(3)
  Fcn4 : Fcn  Expr=u(1)*u(2)*u(3)+u(4)*u(6)
  Fcn5 : Fcn  Expr=u(4)*u(2)*u(3)-u(1)*u(6)
  Fcn6 : Fcn  Expr=u(4)*u(5)
  Fcn7 : Fcn  Expr=u(1)*u(5)
  Fcn8 : Fcn  Expr=-u(2)
  Math Function : Math  Operator=transpose
  Mux1 : Mux  Inputs=2
  Mux2 : Mux  Inputs=9
  Reshape : Reshape  OutputDimensionality=Customize  OutputDimensions=[3,3]
  Trigonometric Function : Trigonometry  Operator=sincos
  LBE : Outport
  wires:
  Mux2/1 -> Reshape/1
  Trigonometric Function/1 -> Mux1/1
  Fcn1/1 -> Mux2/2
  Fcn8/1 -> Mux2/7
  Fcn5/1 -> Mux2/6
  Reshape/1 -> Math Function/1
  EulerAngles_rad/1 -> Trigonometric Function/1
  Fcn7/1 -> Mux2/8
  Fcn/1 -> Mux2/1
  Math Function/1 -> LBE/1  "LBE"
  Fcn4/1 -> Mux2/5
  Mux1/1 -> Fcn/1, Fcn1/1, Fcn2/1, Fcn3/1, Fcn6/1, Fcn7/1, Fcn8/1, Fcn5/1, Fcn4/1
  Trigonometric Function/2 -> Mux1/2
  Fcn3/1 -> Mux2/4
  Fcn2/1 -> Mux2/3
  Fcn6/1 -> Mux2/9
